simulink library "mec_pointmass_generic_ATvoith_DIWA_NXT"  (R2016a)
settings: Solver=ode45  SolverMode=SingleTasking  StartTime=0.0  StopTime=10.0  RelTol=1e-3
undefined symbols (not defined in the file): sMP
(part 2 of 4)

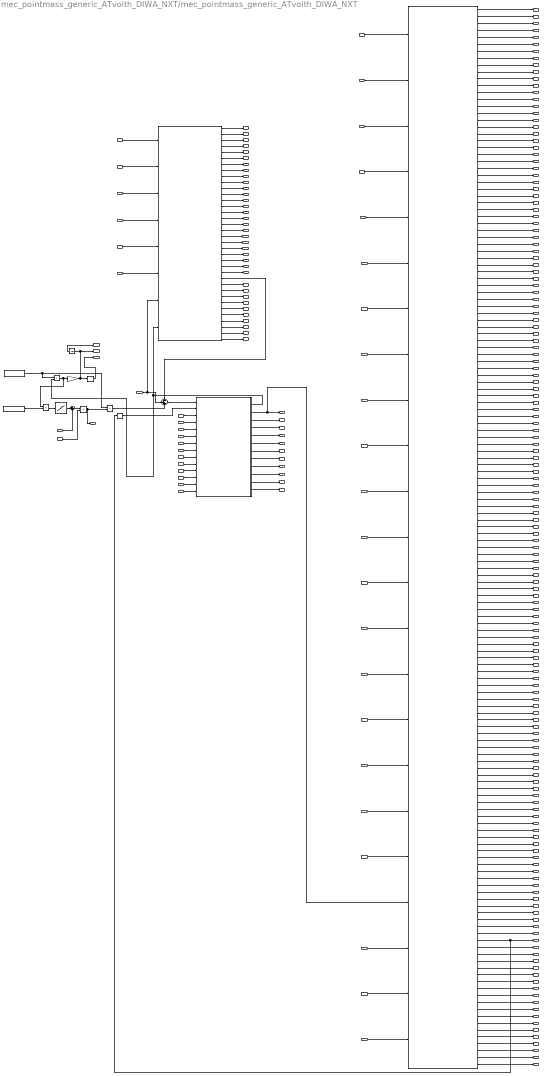
== system mec_pointmass_generic_ATvoith_DIWA_NXT/mec_pointmass_generic_ATvoith_DIWA_NXT  ==
  tcm_AKc2 : Inport
  mec_eng_CrankMean_torque : Inport  Port=2
  tcm_p_EK : Inport  Port=3
  tcm_p_DK : Inport  Port=4
  tcm_p_SK : Inport  Port=5
  tcm_p_PB : Inport  Port=6
  tcm_p_TWB : Inport  Port=7
  tcm_p_TGB : Inport  Port=8
  tcm_AKs2 : Inport  Port=9
  cpc_cdA_offset : Inport  Port=10
  env_curv_pm : Inport  Port=11
  env_density : Inport  Port=12
  env_road_slope_pct : Inport  Port=13
  mec_brk_Axle1_left_torque : Inport  Port=14
  mec_brk_Axle1_right_torque : Inport  Port=15
  mec_brk_Axle2_left_torque : Inport  Port=16
  mec_brk_Axle2_right_torque : Inport  Port=17
  mec_brk_Axle3_left_torque : Inport  Port=18
  mec_brk_Axle3_right_torque : Inport  Port=19
  mec_brk_Axle4_left_torque : Inport  Port=20
  mec_brk_Axle4_right_torque : Inport  Port=21
  mec_brk_TrailerAxle1_left_torque : Inport  Port=22
  mec_brk_TrailerAxle1_right_torque : Inport  Port=23
  mec_brk_TrailerAxle2_left_torque : Inport  Port=24
  mec_brk_TrailerAxle2_right_torque : Inport  Port=25
  mec_brk_TrailerAxle3_left_torque : Inport  Port=26
  mec_brk_TrailerAxle3_right_torque : Inport  Port=27
  mec_ret_Retarder_torque : Inport  Port=28
  mec_veh_GenericLoss_force : Inport  Port=29
  mec_wheel_GenericLoss_torque : Inport  Port=30
  mcm_starter_on : Inport  Port=31
  mec_eng_Starter_torque : Inport  Port=32
  mec_brk_AirCompressor_torque : Inport  Port=33
  mec_eng_Generator_torque : Inport  Port=34
  mec_eng_Consumer_torque : Inport  Port=35
  mec_eng_MainFan_torque : Inport  Port=36
  mec_eng_MainPump_torque : Inport  Port=37
  mec_eng_EmotCrankshaft_torque : Inport  Port=38
  tcm_p_RGK : Inport  Port=39
  pt_RetTrq_Rq_PT : Inport  Port=40
  tcm_gearAct : Inport  Port=41
  pt_ReqGr_Stat_PT : Inport  Port=42
  env_load_massdiff : Inport  Port=43
  Constant : Constant  Value=scalAngVelStarter
  Constant1 : Constant  Value=iStarter
  DIWA_NXT : Subsystem  mask{DIWA_BB_ParNames=sMP.phys.mec.tx.DIWA_BB_ParNames, DIWA_BB_ParValues=sMP.phys.mec.tx.DIWA_BB_ParValues}
  Derivative2 : Derivative
  Engine : Subsystem
  Gain1 : Gain  Gain=pi/30
  Integrator : Integrator
  Memory : Memory
  Product{,1..3} (4 alike) : Product
  StarterMap : Lookup_n-D  NumberOfTableDimensions=1  BreakpointsForDimension1=[0,2.7027,64.8648,150.4214,260.724,378.378,520.398,657.98,819.858,982.04,1178.378,1286.486,1430.18,1578.378,1789.894,2054.06,2177.6,2616.22,3124.32,3697.3,3757.62]  Table=[319.835,318.919,297.838,271.351,244.364,217.585,191.073,165.144,136.757,109.189,82.9584,69.8576,56.7568,44.1906,32.1593,19.8695,15.6757,7.2814,3.27928,0,0]  InternalRulePriority=Speed  RndMeth=Simplest  InputSameDT=on
  Sum : Sum  Inputs=|++
  Sum1 : Sum  Inputs=-++
  mec_pointmass_generic_ATvoith_std : Subsystem  mask{s1=sMP.phys.mec.settings_iMode, s2=sMP.phys.mec.settings_dt, initCmd='Parameters_mec_pointmass_generic_ATvoith_std_sf', p1=sMP.phys.mec.axle1.iDiff, p2=sMP.phys.mec.axle1.isDriven, p3=sMP.phys.mec.axle1.isRearAxle, p4=sMP.phys.mec.brk1.JBrakeDisc_kgm2, p5=sMP.phys.mec.brk1.JHub_kgm2, p6=sMP.phys.mec.axle1.JSideShft_kgm2, p7=sMP.phys.mec.axle2.iDiff, p8=sMP.phys.mec.axle2.isDriven, p9=sMP.phys.mec.axle2.isRearAxle, p10=sMP.phys.mec.brk2.JBrakeDisc_kgm2, p11=sMP.phys.mec.brk2.JHub_kgm2, p12=sMP.phys.mec.axle2.JSideShft_kgm2, p13=sMP.phys.mec.axle3.iDiff, p14=sMP.phys.mec.axle3.isDriven, p15=sMP.phys.mec.axle3.isRearAxle, p16=sMP.phys.mec.brk3.JBrakeDisc_kgm2, p17=sMP.phys.mec.brk3.JHub_kgm2, p18=sMP.phys.mec.axle3.JSideShft_kgm2, p19=sMP.phys.mec.axle4.iDiff, p20=sMP.phys.mec.axle4.isDriven, p21=sMP.phys.mec.axle4.isRearAxle, p22=sMP.phys.mec.brk4.JBrakeDisc_kgm2, p23=sMP.phys.mec.brk4.JHub_kgm2, p24=sMP.phys.mec.axle4.JSideShft_kgm2, p25=sMP.phys.mec.in.cpc_cdA_offset, p26=sMP.phys.mec.in.env_curv_pm, p27=sMP.phys.mec.in.env_density, p28=sMP.phys.mec.in.env_load_massdiff, p29=sMP.phys.mec.in.env_road_slope_pct, p30=sMP.phys.mec.out.mec_brk_Axle1_angAcc, p31=sMP.phys.mec.out.mec_brk_Axle1_angPos, p32=sMP.phys.mec.out.mec_brk_Axle1_angVel, p33=sMP.phys.mec.out.mec_brk_Axle1_left_angAcc, p34=sMP.phys.mec.out.mec_brk_Axle1_left_angPos, p35=sMP.phys.mec.out.mec_brk_Axle1_left_angVel, p36=sMP.phys.mec.in.mec_brk_Axle1_left_torque, p37=sMP.phys.mec.out.mec_brk_Axle1_right_angAcc, p38=sMP.phys.mec.out.mec_brk_Axle1_right_angPos, p39=sMP.phys.mec.out.mec_brk_Axle1_right_angVel, p40=sMP.phys.mec.in.mec_brk_Axle1_right_torque, p41=sMP.phys.mec.out.mec_brk_Axle2_angAcc, p42=sMP.phys.mec.out.mec_brk_Axle2_angPos, p43=sMP.phys.mec.out.mec_brk_Axle2_angVel, p44=sMP.phys.mec.out.mec_brk_Axle2_left_angAcc, p45=sMP.phys.mec.out.mec_brk_Axle2_left_angPos, p46=sMP.phys.mec.out.mec_brk_Axle2_left_angVel, p47=sMP.phys.mec.in.mec_brk_Axle2_left_torque, p48=sMP.phys.mec.out.mec_brk_Axle2_right_angAcc, p49=sMP.phys.mec.out.mec_brk_Axle2_right_angPos, p50=sMP.phys.mec.out.mec_brk_Axle2_right_angVel, p51=sMP.phys.mec.in.mec_brk_Axle2_right_torque, p52=sMP.phys.mec.out.mec_brk_Axle3_angAcc, p53=sMP.phys.mec.out.mec_brk_Axle3_angPos, p54=sMP.phys.mec.out.mec_brk_Axle3_angVel, p55=sMP.phys.mec.out.mec_brk_Axle3_left_angAcc, p56=sMP.phys.mec.out.mec_brk_Axle3_left_angPos, p57=sMP.phys.mec.out.mec_brk_Axle3_left_angVel, p58=sMP.phys.mec.in.mec_brk_Axle3_left_torque, p59=sMP.phys.mec.out.mec_brk_Axle3_right_angAcc, p60=sMP.phys.mec.out.mec_brk_Axle3_right_angPos, p61=sMP.phys.mec.out.mec_brk_Axle3_right_angVel, p62=sMP.phys.mec.in.mec_brk_Axle3_right_torque, p63=sMP.phys.mec.out.mec_brk_Axle4_angAcc, p64=sMP.phys.mec.out.mec_brk_Axle4_angPos, p65=sMP.phys.mec.out.mec_brk_Axle4_angVel, p66=sMP.phys.mec.out.mec_brk_Axle4_left_angAcc, p67=sMP.phys.mec.out.mec_brk_Axle4_left_angPos, p68=sMP.phys.mec.out.mec_brk_Axle4_left_angVel, p69=sMP.phys.mec.in.mec_brk_Axle4_left_torque, p70=sMP.phys.mec.out.mec_brk_Axle4_right_angAcc, p71=sMP.phys.mec.out.mec_brk_Axle4_right_angPos, p72=sMP.phys.mec.out.mec_brk_Axle4_right_angVel, p73=sMP.phys.mec.in.mec_brk_Axle4_right_torque, p74=sMP.phys.mec.out.mec_brk_TrailerAxle1_angAcc, p75=sMP.phys.mec.out.mec_brk_TrailerAxle1_angPos, p76=sMP.phys.mec.out.mec_brk_TrailerAxle1_angVel, p77=sMP.phys.mec.out.mec_brk_TrailerAxle1_left_angAcc, p78=sMP.phys.mec.out.mec_brk_TrailerAxle1_left_angPos, p79=sMP.phys.mec.out.mec_brk_TrailerAxle1_left_angVel, p80=sMP.phys.mec.in.mec_brk_TrailerAxle1_left_torque, p81=sMP.phys.mec.out.mec_brk_TrailerAxle1_right_angAcc, p82=sMP.phys.mec.out.mec_brk_TrailerAxle1_right_angPos, p83=sMP.phys.mec.out.mec_brk_TrailerAxle1_right_angVel, p84=sMP.phys.mec.in.mec_brk_TrailerAxle1_right_torque, p85=sMP.phys.mec.out.mec_brk_TrailerAxle2_angAcc, p86=sMP.phys.mec.out.mec_brk_TrailerAxle2_angPos, p87=sMP.phys.mec.out.mec_brk_TrailerAxle2_angVel, p88=sMP.phys.mec.out.mec_brk_TrailerAxle2_left_angAcc, p89=sMP.phys.mec.out.mec_brk_TrailerAxle2_left_angPos, p90=sMP.phys.mec.out.mec_brk_TrailerAxle2_left_angVel, p91=sMP.phys.mec.in.mec_brk_TrailerAxle2_left_torque, p92=sMP.phys.mec.out.mec_brk_TrailerAxle2_right_angAcc, p93=sMP.phys.mec.out.mec_brk_TrailerAxle2_right_angPos, p94=sMP.phys.mec.out.mec_brk_TrailerAxle2_right_angVel, p95=sMP.phys.mec.in.mec_brk_TrailerAxle2_right_torque, p96=sMP.phys.mec.out.mec_brk_TrailerAxle3_angAcc, p97=sMP.phys.mec.out.mec_brk_TrailerAxle3_angPos, p98=sMP.phys.mec.out.mec_brk_TrailerAxle3_angVel, p99=sMP.phys.mec.out.mec_brk_TrailerAxle3_left_angAcc, p100=sMP.phys.mec.out.mec_brk_TrailerAxle3_left_angPos, p101=sMP.phys.mec.out.mec_brk_TrailerAxle3_left_angVel, p102=sMP.phys.mec.in.mec_brk_TrailerAxle3_left_torque, p103=sMP.phys.mec.out.mec_brk_TrailerAxle3_right_angAcc, p104=sMP.phys.mec.out.mec_brk_TrailerAxle3_right_angPos, p105=sMP.phys.mec.out.mec_brk_TrailerAxle3_right_angVel, p106=sMP.phys.mec.in.mec_brk_TrailerAxle3_right_torque, p107=sMP.phys.mec.in.mec_eng_CrankMean_torque, p108=sMP.phys.mec.out.mec_ret_Retarder_angAcc, p109=sMP.phys.mec.out.mec_ret_Retarder_angPos, p110=sMP.phys.mec.out.mec_ret_Retarder_angVel, p111=sMP.phys.mec.in.mec_ret_Retarder_torque, p112=sMP.phys.mec.out.mec_tx_inclRoadSns, p113=sMP.phys.mec.out.mec_tx_nGbOutD3Sns, p114=sMP.phys.mec.out.mec_tx_nGbOutDzAwSns, p115=sMP.phys.mec.out.mec_tx_nGbOutDzSfSns, p116=sMP.phys.mec.out.mec_tx_nGbOutDzTuAwSns, p117=sMP.phys.mec.out.mec_tx_nGbOutSns, p118=sMP.phys.mec.out.mec_veh_AxleLoad1, p119=sMP.phys.mec.out.mec_veh_AxleLoad2, p120=sMP.phys.mec.out.mec_veh_AxleLoad3, p121=sMP.phys.mec.out.mec_veh_AxleLoad4, p122=sMP.phys.mec.out.mec_veh_fRollCoeffOverall, p123=sMP.phys.mec.in.mec_veh_GenericLoss_force, p124=sMP.phys.mec.out.mec_veh_GenericLoss_transAcc, p125=sMP.phys.mec.out.mec_veh_GenericLoss_transPos, p126=sMP.phys.mec.out.mec_veh_GenericLoss_transVel, p127=sMP.phys.mec.out.mec_veh_massVehicle, p128=sMP.phys.mec.out.mec_veh_Payload, p129=sMP.phys.mec.out.mec_veh_TotalGroCombWeight, p130=sMP.phys.mec.out.mec_veh_TrailerAxleLoad1, p131=sMP.phys.mec.out.mec_veh_TrailerAxleLoad2, p132=sMP.phys.mec.out.mec_veh_TrailerAxleLoad3, p133=sMP.phys.mec.out.mec_veh_transAcc, p134=sMP.phys.mec.out.mec_veh_transPos, p135=sMP.phys.mec.out.mec_veh_transVel, p136=sMP.phys.mec.out.mec_veh_VehVelReferenceCool_velocity, p137=sMP.phys.mec.out.mec_veh_VehVelReferenceUhood_velocity, p138=sMP.phys.mec.out.mec_wheel_GenericLoss_angAcc, p139=sMP.phys.mec.out.mec_wheel_GenericLoss_angPos, p140=sMP.phys.mec.out.mec_wheel_GenericLoss_angVel, p141=sMP.phys.mec.in.mec_wheel_GenericLoss_torque, p142=sMP.phys.mec.out.mec_brk_Axle1_omBrk_info, p143=sMP.phys.mec.out.mec_brk_Axle1_omIn_info, p144=sMP.phys.mec.out.mec_brk_Axle1_TiBrk_info, p145=sMP.phys.mec.out.mec_brk_Axle1_TiLoss_info, p146=sMP.phys.mec.out.mec_brk_Axle1_TIn_info, p147=sMP.phys.mec.out.mec_brk_Axle2_omIn_info, p148=sMP.phys.mec.out.mec_brk_Axle2_TiBrk_info, p149=sMP.phys.mec.out.mec_brk_Axle2_TiLoss_info, p150=sMP.phys.mec.out.mec_brk_Axle2_TIn_info, p151=sMP.phys.mec.out.mec_brk_Axle3_omIn_info, p152=sMP.phys.mec.out.mec_brk_Axle3_TiBrk_info, p153=sMP.phys.mec.out.mec_brk_Axle3_TiLoss_info, p154=sMP.phys.mec.out.mec_brk_Axle3_TIn_info, p155=sMP.phys.mec.out.mec_brk_Axle4_omIn_info, p156=sMP.phys.mec.out.mec_brk_Axle4_TiBrk_info, p157=sMP.phys.mec.out.mec_brk_Axle4_TiLoss_info, p158=sMP.phys.mec.out.mec_brk_Axle4_TIn_info, p159=sMP.phys.mec.out.mec_brk_TrailerAxle1_omIn_info, p160=sMP.phys.mec.out.mec_brk_TrailerAxle1_TiBrk_info, p161=sMP.phys.mec.out.mec_brk_TrailerAxle1_TiLoss_info, p162=sMP.phys.mec.out.mec_brk_TrailerAxle1_TIn_info, p163=sMP.phys.mec.out.mec_brk_TrailerAxle2_omIn_info, p164=sMP.phys.mec.out.mec_brk_TrailerAxle2_TiBrk_info, p165=sMP.phys.mec.out.mec_brk_TrailerAxle2_TiLoss_info, p166=sMP.phys.mec.out.mec_brk_TrailerAxle2_TIn_info, p167=sMP.phys.mec.out.mec_brk_TrailerAxle3_omIn_info, p168=sMP.phys.mec.out.mec_brk_TrailerAxle3_TiBrk_info, p169=sMP.phys.mec.out.mec_brk_TrailerAxle3_TiLoss_info, p170=sMP.phys.mec.out.mec_brk_TrailerAxle3_TIn_info, p171=sMP.phys.mec.out.mec_brk_TrailerWheel1_TiLossRollRes_info, p172=sMP.phys.mec.out.mec_brk_TrailerWheel2_TiLossRollRes_info, p173=sMP.phys.mec.out.mec_brk_TrailerWheel3_TiLossRollRes_info, p174=sMP.phys.mec.out.mec_brk_Wheel1_TiLossRollRes_info, p175=sMP.phys.mec.out.mec_brk_Wheel2_TiLossRollRes_info, p176=sMP.phys.mec.out.mec_brk_Wheel3_TiLossRollRes_info, p177=sMP.phys.mec.out.mec_brk_Wheel4_TiLossRollRes_info, p178=sMP.phys.mec.out.mec_ret_T_info, p179=sMP.phys.mec.out.mec_sht_omShtF_info, p180=sMP.phys.mec.out.mec_sht_omShtR_info, p181=sMP.phys.mec.out.mec_sht_TiLossShtF_info, p182=sMP.phys.mec.out.mec_sht_TiLossShtR_info, p183=sMP.phys.mec.out.mec_tfc_omOut_info, p184=sMP.phys.mec.out.mec_tfc_TiLoss_info, p185=sMP.phys.mec.out.mec_tfc_TOutFront_info, p186=sMP.phys.mec.out.mec_tfc_TOutRear_info, p187=sMP.phys.mec.out.mec_veh_domFW_info, p188=sMP.phys.mec.out.mec_veh_dphiFW_info, p189=sMP.phys.mec.out.mec_veh_FiAirDrag_info, p190=sMP.phys.mec.out.mec_veh_FiGradeRes_info, p191=sMP.phys.mec.out.mec_veh_FWheelTraction_info, p192=sMP.phys.mec.out.mec_veh_sFW_info, p193=sMP.phys.mec.out.mec_veh_TiFW_info, p194=sMP.phys.mec.out.mec_veh_vehConfig_info, p195=sMP.phys.mec.out.mec_wheel_Axle1_T_info, p196=sMP.phys.mec.out.mec_wheel_Axle2_T_info, p197=sMP.phys.mec.out.mec_wheel_Axle3_T_info, p198=sMP.phys.mec.out.mec_wheel_Axle4_T_info, p199=sMP.phys.mec.out.mec_wheel_TrailerAxle1_T_info, p200=sMP.phys.mec.out.mec_wheel_TrailerAxle2_T_info, p201=sMP.phys.mec.out.mec_wheel_TrailerAxle3_T_info, p202=sMP.phys.mec.shtF.JPropShaft_kgm2, p203=sMP.phys.mec.shtR.JPropShaft_kgm2, p204=sMP.phys.mec.ret.iRet, p205=sMP.phys.mec.ret.JRet_kgm2, p206=sMP.phys.mec.ret.JRetdrvgear_kgm2, p207=sMP.phys.mec.trailerAxle1.iDiff, p208=sMP.phys.mec.trailerAxle1.isDriven, p209=sMP.phys.mec.trailerAxle1.isRearAxle, p210=sMP.phys.mec.trailerBrk1.JBrakeDisc_kgm2, p211=sMP.phys.mec.trailerBrk1.JHub_kgm2, p212=sMP.phys.mec.trailerAxle1.JSideShft_kgm2, p213=sMP.phys.mec.trailerAxle2.iDiff, p214=sMP.phys.mec.trailerAxle2.isDriven, p215=sMP.phys.mec.trailerAxle2.isRearAxle, p216=sMP.phys.mec.trailerBrk2.JBrakeDisc_kgm2, p217=sMP.phys.mec.trailerBrk2.JHub_kgm2, p218=sMP.phys.mec.trailerAxle2.JSideShft_kgm2, p219=sMP.phys.mec.trailerAxle3.iDiff, p220=sMP.phys.mec.trailerAxle3.isDriven, p221=sMP.phys.mec.trailerAxle3.isRearAxle, p222=sMP.phys.mec.trailerBrk3.JBrakeDisc_kgm2, p223=sMP.phys.mec.trailerBrk3.JHub_kgm2, p224=sMP.phys.mec.trailerAxle3.JSideShft_kgm2, p225=sMP.phys.mec.tfc.JTfc_kgm2, p226=sMP.phys.mec.tfc.stTrfGrBoxHi, p227=sMP.phys.mec.aero.aeroCdA_m2, p228=sMP.phys.mec.aero.aeroRhoAirDensity_kgpm3, p229=sMP.phys.mec.massLoad.number_of_weights, p230=sMP.phys.mec.mass.startGCW_kg, p231=sMP.phys.mec.wheel1.fRollCoeff, p232=sMP.phys.mec.wheel1.JWheel_kgm2, p233=sMP.phys.mec.wheel1.rDyn_m, p234=sMP.phys.mec.wheel2.fRollCoeff, p235=sMP.phys.mec.wheel2.JWheel_kgm2, p236=sMP.phys.mec.wheel2.rDyn_m, p237=sMP.phys.mec.wheel3.fRollCoeff, p238=sMP.phys.mec.wheel3.JWheel_kgm2, p239=sMP.phys.mec.wheel3.rDyn_m, p240=sMP.phys.mec.wheel4.fRollCoeff, p241=sMP.phys.mec.wheel4.JWheel_kgm2, p242=sMP.phys.mec.wheel4.rDyn_m, p243=sMP.phys.mec.trailerWheel1.fRollCoeff, p244=sMP.phys.mec.trailerWheel1.JWheel_kgm2, p245=sMP.phys.mec.trailerWheel1.rDyn_m, p246=sMP.phys.mec.trailerWheel2.fRollCoeff, p247=sMP.phys.mec.trailerWheel2.JWheel_kgm2, p248=sMP.phys.mec.trailerWheel2.rDyn_m, p249=sMP.phys.mec.trailerWheel3.fRollCoeff, p250=sMP.phys.mec.trailerWheel3.JWheel_kgm2, p251=sMP.phys.mec.trailerWheel3.rDyn_m, p252=sMP.phys.mec.mecConsumers.genericWheelLoss_dim, p253=sMP.phys.mec.mecConsumers.genericVehicleLoss_dim, p254=sMP.phys.mec.axle1.axleLoss_dim, p255=sMP.phys.mec.axle1.axleLoss_map_torqueAxleIn_Nm, p256=sMP.phys.mec.axle1.axleLoss_x_speedAxleOut_rpm, p257=sMP.phys.mec.axle1.axleLoss_y_torqueAxleIn_Nm, p258=sMP.phys.mec.axle2.axleLoss_dim, p259=sMP.phys.mec.axle2.axleLoss_map_torqueAxleIn_Nm, p260=sMP.phys.mec.axle2.axleLoss_x_speedAxleOut_rpm, p261=sMP.phys.mec.axle2.axleLoss_y_torqueAxleIn_Nm, p262=sMP.phys.mec.axle3.axleLoss_dim, p263=sMP.phys.mec.axle3.axleLoss_map_torqueAxleIn_Nm, p264=sMP.phys.mec.axle3.axleLoss_x_speedAxleOut_rpm, p265=sMP.phys.mec.axle3.axleLoss_y_torqueAxleIn_Nm, p266=sMP.phys.mec.axle4.axleLoss_dim, p267=sMP.phys.mec.axle4.axleLoss_map_torqueAxleIn_Nm, p268=sMP.phys.mec.axle4.axleLoss_x_speedAxleOut_rpm, p269=sMP.phys.mec.axle4.axleLoss_y_torqueAxleIn_Nm, p270=sMP.phys.mec.shtF.shtLoss_dim, p271=sMP.phys.mec.shtF.shtLoss_map_torqueShtIn_Nm, p272=sMP.phys.mec.shtF.shtLoss_x_speedShtIn_rpm, p273=sMP.phys.mec.shtF.shtLoss_y_torqueShtIn_Nm, p274=sMP.phys.mec.shtR.shtLoss_dim, p275=sMP.phys.mec.shtR.shtLoss_map_torqueShtIn_Nm, p276=sMP.phys.mec.shtR.shtLoss_x_speedShtIn_rpm, p277=sMP.phys.mec.shtR.shtLoss_y_torqueShtIn_Nm, p278=sMP.phys.mec.trailerAxle1.axleLoss_dim, p279=sMP.phys.mec.trailerAxle1.axleLoss_map_torqueAxleIn_Nm, p280=sMP.phys.mec.trailerAxle1.axleLoss_x_speedAxleOut_rpm, p281=sMP.phys.mec.trailerAxle1.axleLoss_y_torqueAxleIn_Nm, p282=sMP.phys.mec.trailerAxle2.axleLoss_dim, p283=sMP.phys.mec.trailerAxle2.axleLoss_map_torqueAxleIn_Nm, p284=sMP.phys.mec.trailerAxle2.axleLoss_x_speedAxleOut_rpm, p285=sMP.phys.mec.trailerAxle2.axleLoss_y_torqueAxleIn_Nm, p286=sMP.phys.mec.trailerAxle3.axleLoss_dim, p287=sMP.phys.mec.trailerAxle3.axleLoss_map_torqueAxleIn_Nm, p288=sMP.phys.mec.trailerAxle3.axleLoss_x_speedAxleOut_rpm, p289=sMP.phys.mec.trailerAxle3.axleLoss_y_torqueAxleIn_Nm, p290=sMP.phys.mec.tfc.iTfc, p291=sMP.phys.mec.tfc.tfcLoss_dim, p292=sMP.phys.mec.tfc.tfcLoss_map_torqueTfcIn_Nm, p293=sMP.phys.mec.tfc.tfcLoss_x_speedTfcIn_rpm, p294=sMP.phys.mec.tfc.tfcLoss_y_torqueTfcIn_Nm, p295=sMP.phys.mec.tfc.torqueDistribution, p296=sMP.phys.mec.massLoad.mass_distribution, p297=sMP.phys.mec.mecConsumers.genericWheelLoss_x_speed_rpm, p298=sMP.phys.mec.mecConsumers.genericWheelLoss_map_lossTorque_Nm, p299=sMP.phys.mec.mecConsumers.genericVehicleLoss_x_velocity_kmh, p300=sMP.phys.mec.mecConsumers.genericVehicleLoss_map_loss_N}
      mask prompts: s1 "Solver Type: settings_iMode [-]"; s2 "Solver Step Size: settings_dt [s]"; initCmd "Initialization command"; p1 "Ratio Differential Gear [-] export=true name=iDiff prio=1 dataSetName=axle_dummy dataClassType=axle dataClassName=$dataClassNameAxle$ moduleXmlReference=$moduleXmlReferenceAxle$ unit='-' description='Ratio Differential Gear': axle1.iDiff [-]"; p2 "Is driven Axle? [-] export=true name=isDriven prio=1 dataSetName=axle_dummy dataClassType=axle dataClassName=$dataClassNameAxle$ moduleXmlReference=$moduleXmlReferenceAxle$ unit='-' description='Is Driven Axle': axle1.isDriven [-]"; p3 "Is rear Axle? [-] export=true name=isRearAxle prio=1 dataSetName=axle_dummy dataClassType=axle dataClassName=$dataClassNameAxle$ moduleXmlReference=$moduleXmlReferenceAxle$ unit='-' description='Is Rear Axle': axle1.isRearAxle [-]"; p4 "Inertia Brake Disc  [kgm^2] export=true name=JBrakeDisc_kgm2 prio=1 dataSetName=brk_dummy dataClassType=brk dataClassName=$dataClassNameBrk$ moduleXmlReference=$moduleXmlReferenceBrk$ unit='kgm^2' description='Inertia Brake Disc': axle1.JBrakeDisc_kgm2 [kgm²]"; p5 "Inertia Hub  [kgm^2] export=true name=JHub_kgm2 prio=1 dataSetName=brk_dummy dataClassType=brk dataClassName=$dataClassNameBrk$ moduleXmlReference=$moduleXmlReferenceBrk$ unit='kgm^2' description='Inertia Hub': axle1.JHub_kgm2 [-]"; p6 "Inertia Side Shaft [kgm^2] export=true name=JSideShft_kgm2 prio=1 dataSetName=axle_dummy dataClassType=axle dataClassName=$dataClassNameAxle$ moduleXmlReference=$moduleXmlReferenceAxle$ unit='kgm^2' description='Inertia Side Shaft': axle1.JSideShft_kgm2 [kgm²]"; p7 "Ratio Differential Gear [-] export=true name=iDiff prio=1 dataSetName=axle_dummy dataClassType=axle dataClassName=$dataClassNameAxle$ moduleXmlReference=$moduleXmlReferenceAxle$ unit='-' description='Ratio Differential Gear': axle2.iDiff [-]"; p8 "Is driven Axle? [-] export=true name=isDriven prio=1 dataSetName=axle_dummy dataClassType=axle dataClassName=$dataClassNameAxle$ moduleXmlReference=$moduleXmlReferenceAxle$ unit='-' description='Is Driven Axle': axle2.isDriven [-]"; p9 "Is rear Axle? [-] export=true name=isRearAxle prio=1 dataSetName=axle_dummy dataClassType=axle dataClassName=$dataClassNameAxle$ moduleXmlReference=$moduleXmlReferenceAxle$ unit='-' description='Is Rear Axle': axle2.isRearAxle [-]"; p10 "Inertia Brake Disc  [kgm^2] export=true name=JBrakeDisc_kgm2 prio=1 dataSetName=brk_dummy dataClassType=brk dataClassName=$dataClassNameBrk$ moduleXmlReference=$moduleXmlReferenceBrk$ unit='kgm^2' description='Inertia Brake Disc': axle2.JBrakeDisc_kgm2 [kgm²]"; p11 "Inertia Hub  [kgm^2] export=true name=JHub_kgm2 prio=1 dataSetName=brk_dummy dataClassType=brk dataClassName=$dataClassNameBrk$ moduleXmlReference=$moduleXmlReferenceBrk$ unit='kgm^2' description='Inertia Hub': axle2.JHub_kgm2 [-]"; p12 "Inertia Side Shaft [kgm^2] export=true name=JSideShft_kgm2 prio=1 dataSetName=axle_dummy dataClassType=axle dataClassName=$dataClassNameAxle$ moduleXmlReference=$moduleXmlReferenceAxle$ unit='kgm^2' description='Inertia Side Shaft': axle2.JSideShft_kgm2 [kgm²]"; p13 "Ratio Differential Gear [-] export=true name=iDiff prio=1 dataSetName=axle_dummy dataClassType=axle dataClassName=$dataClassNameAxle$ moduleXmlReference=$moduleXmlReferenceAxle$ unit='-' description='Ratio Differential Gear': axle3.iDiff [-]"; p14 "Is driven Axle? [-] export=true name=isDriven prio=1 dataSetName=axle_dummy dataClassType=axle dataClassName=$dataClassNameAxle$ moduleXmlReference=$moduleXmlReferenceAxle$ unit='-' description='Is Driven Axle': axle3.isDriven [-]"; p15 "Is rear Axle? [-] export=true name=isRearAxle prio=1 dataSetName=axle_dummy dataClassType=axle dataClassName=$dataClassNameAxle$ moduleXmlReference=$moduleXmlReferenceAxle$ unit='-' description='Is Rear Axle': axle3.isRearAxle [-]"; p16 "Inertia Brake Disc  [kgm^2] export=true name=JBrakeDisc_kgm2 prio=1 dataSetName=brk_dummy dataClassType=brk dataClassName=$dataClassNameBrk$ moduleXmlReference=$moduleXmlReferenceBrk$ unit='kgm^2' description='Inertia Brake Disc': axle3.JBrakeDisc_kgm2 [kgm²]"; p17 "Inertia Hub  [kgm^2] export=true name=JHub_kgm2 prio=1 dataSetName=brk_dummy dataClassType=brk dataClassName=$dataClassNameBrk$ moduleXmlReference=$moduleXmlReferenceBrk$ unit='kgm^2' description='Inertia Hub': axle3.JHub_kgm2 [-]"; p18 "Inertia Side Shaft [kgm^2] export=true name=JSideShft_kgm2 prio=1 dataSetName=axle_dummy dataClassType=axle dataClassName=$dataClassNameAxle$ moduleXmlReference=$moduleXmlReferenceAxle$ unit='kgm^2' description='Inertia Side Shaft': axle3.JSideShft_kgm2 [kgm²]"; p19 "Ratio Differential Gear [-] export=true name=iDiff prio=1 dataSetName=axle_dummy dataClassType=axle dataClassName=$dataClassNameAxle$ moduleXmlReference=$moduleXmlReferenceAxle$ unit='-' description='Ratio Differential Gear': axle4.iDiff [-]"; p20 "Is driven Axle? [-] export=true name=isDriven prio=1 dataSetName=axle_dummy dataClassType=axle dataClassName=$dataClassNameAxle$ moduleXmlReference=$moduleXmlReferenceAxle$ unit='-' description='Is Driven Axle': axle4.isDriven [-]"; p21 "Is rear Axle? [-] export=true name=isRearAxle prio=1 dataSetName=axle_dummy dataClassType=axle dataClassName=$dataClassNameAxle$ moduleXmlReference=$moduleXmlReferenceAxle$ unit='-' description='Is Rear Axle': axle4.isRearAxle [-]"; p22 "Inertia Brake Disc  [kgm^2] export=true name=JBrakeDisc_kgm2 prio=1 dataSetName=brk_dummy dataClassType=brk dataClassName=$dataClassNameBrk$ moduleXmlReference=$moduleXmlReferenceBrk$ unit='kgm^2' description='Inertia Brake Disc': axle4.JBrakeDisc_kgm2 [kgm²]"; p23 "Inertia Hub  [kgm^2] export=true name=JHub_kgm2 prio=1 dataSetName=brk_dummy dataClassType=brk dataClassName=$dataClassNameBrk$ moduleXmlReference=$moduleXmlReferenceBrk$ unit='kgm^2' description='Inertia Hub': axle4.JHub_kgm2 [-]"; p24 "Inertia Side Shaft [kgm^2] export=true name=JSideShft_kgm2 prio=1 dataSetName=axle_dummy dataClassType=axle dataClassName=$dataClassNameAxle$ moduleXmlReference=$moduleXmlReferenceAxle$ unit='kgm^2' description='Inertia Side Shaft': axle4.JSideShft_kgm2 [kgm²]"; p25 "Additive Controlable Air Resistance (init) export=$sw_cpc_cdA_offset$ name=cpc_cdA_offset prio=1 dataSetName=std dataClassType=initIO dataClassName=initIO unit='' description='Additive Controlable Air Resistance': interface_IO.cpc_cdA_offset_0 [-]"; p26 "Curve Curvature (init) export=$sw_env_curv_pm$ name=env_curv_pm prio=1 dataSetName=std dataClassType=initIO dataClassName=initIO unit='1/m' description='Curve Curvature': interface_IO.env_curv_pm_0 [-]"; p27 "Air density from environment (init) export=$sw_env_density$ name=env_density prio=1 dataSetName=std dataClassType=initIO dataClassName=initIO unit='kg/m^3' description='Air density from environment': interface_IO.env_density_0 [-]"; p28 "Mass Difference (init) export=$sw_env_load_massdiff$ name=env_load_massdiff prio=1 dataSetName=std dataClassType=initIO dataClassName=initIO unit='1/m' description='Curve Curvature': interface_IO.env_load_massdiff_0 [-]"; p29 "Slope of road from environment (init) export=$sw_env_road_slope_pct$ name=env_road_slope_pct prio=1 dataSetName=std dataClassType=initIO dataClassName=initIO unit='-' description='Slope of road from environment': interface_IO.env_road_slope_pct_0 [-]"; p30 "Acceleration Brake 1 (init) export=$sw_mec_brk_Axle1_angAcc$ name=mec_brk_Axle1_angAcc prio=1 dataSetName=std dataClassType=initIO dataClassName=initIO unit='rad/s^2' description='Acceleration Brake 1': interface_IO.mec_brk_Axle1_angAcc_0 [-]"; p31 "Angle Brake 1 (init) export=$sw_mec_brk_Axle1_angPos$ name=mec_brk_Axle1_angPos prio=1 dataSetName=std dataClassType=initIO dataClassName=initIO unit='rad' description='Angle Brake 1': interface_IO.mec_brk_Axle1_angPos_0 [-]"; p32 "Velocity Brake 1 (init) export=$sw_mec_brk_Axle1_angVel$ name=mec_brk_Axle1_angVel prio=1 dataSetName=std dataClassType=initIO dataClassName=initIO unit='rad/s' description='Velocity Brake 1': interface_IO.mec_brk_Axle1_angVel_0 [-]"; p33 "Acceleration Brake 1 left Wheel (init) export=$sw_mec_brk_Axle1_left_angAcc$ name=mec_brk_Axle1_left_angAcc prio=1 dataSetName=std dataClassType=initIO dataClassName=initIO unit='rad/s^2' description='Acceleration Brake 1 left Wheel': interface_IO.mec_brk_Axle1_left_angAcc_0 [-]"; p34 "Angle Brake 1 left Wheel (init) export=$sw_mec_brk_Axle1_left_angPos$ name=mec_brk_Axle1_left_angPos prio=1 dataSetName=std dataClassType=initIO dataClassName=initIO unit='rad' description='Angle Brake 1 left Wheel': interface_IO.mec_brk_Axle1_left_angPos_0 [-]"; p35 "Velocity Brake 1 left Wheel (init) export=$sw_mec_brk_Axle1_left_angVel$ name=mec_brk_Axle1_left_angVel prio=1 dataSetName=std dataClassType=initIO dataClassName=initIO unit='rad/s' description='Velocity Brake 1 left Wheel': interface_IO.mec_brk_Axle1_left_angVel_0 [-]"; p36 "Torque Brake 1 left Wheel (init) export=$sw_mec_brk_Axle1_left_torque$ name=mec_brk_Axle1_left_torque prio=1 dataSetName=std dataClassType=initIO dataClassName=initIO unit='Nm' description='Torque Brake 1 left Wheel': interface_IO.mec_brk_Axle1_left_torque_0 [-]"; p37 "Acceleration Brake 1 right Wheel (init) export=$sw_mec_brk_Axle1_right_angAcc$ name=mec_brk_Axle1_right_angAcc prio=1 dataSetName=std dataClassType=initIO dataClassName=initIO unit='rad/s^2' description='Acceleration Brake 1 right Wheel': interface_IO.mec_brk_Axle1_right_angAcc_0 [-]"; p38 "Angle Brake 1 right Wheel (init) export=$sw_mec_brk_Axle1_right_angPos$ name=mec_brk_Axle1_right_angPos prio=1 dataSetName=std dataClassType=initIO dataClassName=initIO unit='rad' description='Angle Brake 1 right Wheel': interface_IO.mec_brk_Axle1_right_angPos_0 [-]"; p39 "Velocity Brake 1 right Wheel (init) export=$sw_mec_brk_Axle1_right_angVel$ name=mec_brk_Axle1_right_angVel prio=1 dataSetName=std dataClassType=initIO dataClassName=initIO unit='rad/s' description='Velocity Brake 1 right Wheel': interface_IO.mec_brk_Axle1_right_angVel_0 [-]"; p40 "Torque Brake 1 left Wheel (init) export=$sw_mec_brk_Axle1_right_torque$ name=mec_brk_Axle1_right_torque prio=1 dataSetName=std dataClassType=initIO dataClassName=initIO unit='Nm' description='Torque Brake 1 left Wheel': interface_IO.mec_brk_Axle1_right_torque_0 [-]"; p41 "Acceleration Brake 2 (init) export=$sw_mec_brk_Axle2_angAcc$ name=mec_brk_Axle2_angAcc prio=1 dataSetName=std dataClassType=initIO dataClassName=initIO unit='rad/s^2' description='Acceleration Brake 2': interface_IO.mec_brk_Axle2_angAcc_0 [-]"; p42 "Angle Brake 2 (init) export=$sw_mec_brk_Axle2_angPos$ name=mec_brk_Axle2_angPos prio=1 dataSetName=std dataClassType=initIO dataClassName=initIO unit='rad' description='Angle Brake 2': interface_IO.mec_brk_Axle2_angPos_0 [-]"; p43 "Velocity Brake 2 (init) export=$sw_mec_brk_Axle2_angVel$ name=mec_brk_Axle2_angVel prio=1 dataSetName=std dataClassType=initIO dataClassName=initIO unit='rad/s' description='Velocity Brake 3': interface_IO.mec_brk_Axle2_angVel_0 [-]"; p44 "Acceleration Brake 2 left Wheel (init) export=$sw_mec_brk_Axle2_left_angAcc$ name=mec_brk_Axle2_left_angAcc prio=1 dataSetName=std dataClassType=initIO dataClassName=initIO unit='rad/s^2' description='Acceleration Brake 2 left Wheel': interface_IO.mec_brk_Axle2_left_angAcc_0 [-]"; p45 "Angle Brake 2 left Wheel (init) export=$sw_mec_brk_Axle2_left_angPos$ name=mec_brk_Axle2_left_angPos prio=1 dataSetName=std dataClassType=initIO dataClassName=initIO unit='rad' description='Angle Brake 2 left Wheel': interface_IO.mec_brk_Axle2_left_angPos_0 [-]"; p46 "Velocity Brake 2 left Wheel (init) export=$sw_mec_brk_Axle2_left_angVel$ name=mec_brk_Axle2_left_angVel prio=1 dataSetName=std dataClassType=initIO dataClassName=initIO unit='rad/s' description='Velocity Brake 3 left Wheel': interface_IO.mec_brk_Axle2_left_angVel_0 [-]"; p47 "Torque Brake 2 left Wheel (init) export=$sw_mec_brk_Axle2_left_torque$ name=mec_brk_Axle2_left_torque prio=1 dataSetName=std dataClassType=initIO dataClassName=initIO unit='Nm' description='Torque Brake 2 left Wheel': interface_IO.mec_brk_Axle2_left_torque_0 [-]"; p48 "Acceleration Brake 2 right Wheel (init) export=$sw_mec_brk_Axle2_right_angAcc$ name=mec_brk_Axle2_right_angAcc prio=1 dataSetName=std dataClassType=initIO dataClassName=initIO unit='rad/s^2' description='Acceleration Brake 2 right Wheel': interface_IO.mec_brk_Axle2_right_angAcc_0 [-]"; p49 "Angle Brake 2 right Wheel (init) export=$sw_mec_brk_Axle2_right_angPos$ name=mec_brk_Axle2_right_angPos prio=1 dataSetName=std dataClassType=initIO dataClassName=initIO unit='rad' description='Angle Brake 2 right Wheel': interface_IO.mec_brk_Axle2_right_angPos_0 [-]"; p50 "Velocity Brake 2 right Wheel (init) export=$sw_mec_brk_Axle2_right_angVel$ name=mec_brk_Axle2_right_angVel prio=1 dataSetName=std dataClassType=initIO dataClassName=initIO unit='rad/s' description='Velocity Brake 3 right Wheel': interface_IO.mec_brk_Axle2_right_angVel_0 [-]"; p51 "Torque Brake 2 right Wheel (init) export=$sw_mec_brk_Axle2_right_torque$ name=mec_brk_Axle2_right_torque prio=1 dataSetName=std dataClassType=initIO dataClassName=initIO unit='Nm' description='Torque Brake 2 right Wheel': interface_IO.mec_brk_Axle2_right_torque_0 [-]"; p52 "Acceleration Brake 3 (init) export=$sw_mec_brk_Axle3_angAcc$ name=mec_brk_Axle3_angAcc prio=1 dataSetName=std dataClassType=initIO dataClassName=initIO unit='rad/s^2' description='Acceleration Brake 3': interface_IO.mec_brk_Axle3_angAcc_0 [-]"; p53 "Angle Brake 3 (init) export=$sw_mec_brk_Axle3_angPos$ name=mec_brk_Axle3_angPos prio=1 dataSetName=std dataClassType=initIO dataClassName=initIO unit='rad' description='Angle Brake 3': interface_IO.mec_brk_Axle3_angPos_0 [-]"; p54 "Velocity Brake 3 (init) export=$sw_mec_brk_Axle3_angVel$ name=mec_brk_Axle3_angVel prio=1 dataSetName=std dataClassType=initIO dataClassName=initIO unit='rad/s' description='Velocity Brake 3': interface_IO.mec_brk_Axle3_angVel_0 [-]"; p55 "Acceleration Brake 3 left Wheel (init) export=$sw_mec_brk_Axle3_left_angAcc$ name=mec_brk_Axle3_left_angAcc prio=1 dataSetName=std dataClassType=initIO dataClassName=initIO unit='rad/s^2' description='Acceleration Brake 3 left Wheel': interface_IO.mec_brk_Axle3_left_angAcc_0 [-]"; p56 "Angle Brake 3 left Wheel (init) export=$sw_mec_brk_Axle3_left_angPos$ name=mec_brk_Axle3_left_angPos prio=1 dataSetName=std dataClassType=initIO dataClassName=initIO unit='rad' description='Angle Brake 3 left Wheel': interface_IO.mec_brk_Axle3_left_angPos_0 [-]"; p57 "Velocity Brake 3 left Wheel (init) export=$sw_mec_brk_Axle3_left_angVel$ name=mec_brk_Axle3_left_angVel prio=1 dataSetName=std dataClassType=initIO dataClassName=initIO unit='rad/s' description='Velocity Brake 3 left Wheel': interface_IO.mec_brk_Axle3_left_angVel_0 [-]"; p58 "Torque Brake 3 left Wheel (init) export=$sw_mec_brk_Axle3_left_torque$ name=mec_brk_Axle3_left_torque prio=1 dataSetName=std dataClassType=initIO dataClassName=initIO unit='Nm' description='Torque Brake 3 left Wheel': interface_IO.mec_brk_Axle3_left_torque_0 [-]"; p59 "Acceleration Brake 3 right Wheel (init) export=$sw_mec_brk_Axle3_right_angAcc$ name=mec_brk_Axle3_right_angAcc prio=1 dataSetName=std dataClassType=initIO dataClassName=initIO unit='rad/s^2' description='Acceleration Brake 3 right Wheel': interface_IO.mec_brk_Axle3_right_angAcc_0 [-]"; p60 "Angle Brake 3 right Wheel (init) export=$sw_mec_brk_Axle3_right_angPos$ name=mec_brk_Axle3_right_angPos prio=1 dataSetName=std dataClassType=initIO dataClassName=initIO unit='rad' description='Angle Brake 3 right Wheel': interface_IO.mec_brk_Axle3_right_angPos_0 [-]"; p61 "Velocity Brake 3 right Wheel (init) export=$sw_mec_brk_Axle3_right_angVel$ name=mec_brk_Axle3_right_angVel prio=1 dataSetName=std dataClassType=initIO dataClassName=initIO unit='rad/s' description='Velocity Brake 3 right Wheel': interface_IO.mec_brk_Axle3_right_angVel_0 [-]"; p62 "Torque Brake 3 right Wheel (init) export=$sw_mec_brk_Axle3_right_torque$ name=mec_brk_Axle3_right_torque prio=1 dataSetName=std dataClassType=initIO dataClassName=initIO unit='Nm' description='Torque Brake 3 right Wheel': interface_IO.mec_brk_Axle3_right_torque_0 [-]"; p63 "Acceleration Brake 4 (init) export=$sw_mec_brk_Axle4_angAcc$ name=mec_brk_Axle4_angAcc prio=1 dataSetName=std dataClassType=initIO dataClassName=initIO unit='rad/s^2' description='Acceleration Brake 4': interface_IO.mec_brk_Axle4_angAcc_0 [-]"; p64 "Angle Brake 4 (init) export=$sw_mec_brk_Axle4_angPos$ name=mec_brk_Axle4_angPos prio=1 dataSetName=std dataClassType=initIO dataClassName=initIO unit='rad' description='Angle Brake 4': interface_IO.mec_brk_Axle4_angPos_0 [-]"; p65 "Velocity Brake 4 (init) export=$sw_mec_brk_Axle4_angVel$ name=mec_brk_Axle4_angVel prio=1 dataSetName=std dataClassType=initIO dataClassName=initIO unit='rad/s' description='Velocity Brake 4': interface_IO.mec_brk_Axle4_angVel_0 [-]"; p66 "Acceleration Brake 4 left Wheel (init) export=$sw_mec_brk_Axle4_left_angAcc$ name=mec_brk_Axle4_left_angAcc prio=1 dataSetName=std dataClassType=initIO dataClassName=initIO unit='rad/s^2' description='Acceleration Brake 4 left Wheel': interface_IO.mec_brk_Axle4_left_angAcc_0 [-]"; p67 "Angle Brake 4 left Wheel (init) export=$sw_mec_brk_Axle4_left_angPos$ name=mec_brk_Axle4_left_angPos prio=1 dataSetName=std dataClassType=initIO dataClassName=initIO unit='rad' description='Angle Brake 4 left Wheel': interface_IO.mec_brk_Axle4_left_angPos_0 [-]"; p68 "Velocity Brake 4 left Wheel (init) export=$sw_mec_brk_Axle4_left_angVel$ name=mec_brk_Axle4_left_angVel prio=1 dataSetName=std dataClassType=initIO dataClassName=initIO unit='rad/s' description='Velocity Brake 4 left Wheel': interface_IO.mec_brk_Axle4_left_angVel_0 [-]"; p69 "Torque Brake 4 left Wheel (init) export=$sw_mec_brk_Axle4_left_torque$ name=mec_brk_Axle4_left_torque prio=1 dataSetName=std dataClassType=initIO dataClassName=initIO unit='Nm' description='Torque Brake 4 left Wheel': interface_IO.mec_brk_Axle4_left_torque_0 [-]"; p70 "Acceleration Brake 4 right Wheel (init) export=$sw_mec_brk_Axle4_right_angAcc$ name=mec_brk_Axle4_right_angAcc prio=1 dataSetName=std dataClassType=initIO dataClassName=initIO unit='rad/s^2' description='Acceleration Brake 4 right Wheel': interface_IO.mec_brk_Axle4_right_angAcc_0 [-]"; p71 "Angle Brake 4 right Wheel (init) export=$sw_mec_brk_Axle4_right_angPos$ name=mec_brk_Axle4_right_angPos prio=1 dataSetName=std dataClassType=initIO dataClassName=initIO unit='rad' description='Angle Brake 4 right Wheel': interface_IO.mec_brk_Axle4_right_angPos_0 [-]"; p72 "Velocity Brake 4 right Wheel (init) export=$sw_mec_brk_Axle4_right_angVel$ name=mec_brk_Axle4_right_angVel prio=1 dataSetName=std dataClassType=initIO dataClassName=initIO unit='rad/s' description='Velocity Brake 4 right Wheel': interface_IO.mec_brk_Axle4_right_angVel_0 [-]"; p73 "Torque Brake 4 right Wheel (init) export=$sw_mec_brk_Axle4_right_torque$ name=mec_brk_Axle4_right_torque prio=1 dataSetName=std dataClassType=initIO dataClassName=initIO unit='Nm' description='Torque Brake 4 right Wheel': interface_IO.mec_brk_Axle4_right_torque_0 [-]"; p74 "Acceleration Trailer Brake 1 (init) export=$sw_mec_brk_TrailerAxle1_angAcc$ name=mec_brk_TrailerAxle1_angAcc prio=1 dataSetName=std dataClassType=initIO dataClassName=initIO unit='rad/s^2' description='Acceleration Trailer Brake 1': interface_IO.mec_brk_TrailerAxle1_angAcc_0 [-]"; p75 "Angle Trailer Brake 1 (init) export=$sw_mec_brk_TrailerAxle1_angPos$ name=mec_brk_TrailerAxle1_angPos prio=1 dataSetName=std dataClassType=initIO dataClassName=initIO unit='rad' description='Angle Trailer Brake 1': interface_IO.mec_brk_TrailerAxle1_angPos_0 [-]"; p76 "Velocity Trailer Brake 1 (init) export=$sw_mec_brk_TrailerAxle1_angVel$ name=mec_brk_TrailerAxle1_angVel prio=1 dataSetName=std dataClassType=initIO dataClassName=initIO unit='rad/s' description='Velocity Trailer Brake 1': interface_IO.mec_brk_TrailerAxle1_angVel_0 [-]"; p77 "Acceleration Trailer Brake 1 left Wheel (init) export=$sw_mec_brk_TrailerAxle1_left_angAcc$ name=mec_brk_TrailerAxle1_left_angAcc prio=1 dataSetName=std dataClassType=initIO dataClassName=initIO unit='rad/s^2' description='Acceleration Trailer Brake 1 left Wheel': interface_IO.mec_brk_TrailerAxle1_left_angAcc_0 [-]"; p78 "Angle Trailer Brake 1 left Wheel (init) export=$sw_mec_brk_TrailerAxle1_left_angPos$ name=mec_brk_TrailerAxle1_left_angPos prio=1 dataSetName=std dataClassType=initIO dataClassName=initIO unit='rad' description='Angle Trailer Brake 1 left Wheel': interface_IO.mec_brk_TrailerAxle1_left_angPos_0 [-]"; p79 "Velocity Trailer Brake 1 left Wheel (init) export=$sw_mec_brk_TrailerAxle1_left_angVel$ name=mec_brk_TrailerAxle1_left_angVel prio=1 dataSetName=std dataClassType=initIO dataClassName=initIO unit='rad/s' description='Velocity Trailer Brake 1 left Wheel': interface_IO.mec_brk_TrailerAxle1_left_angVel_0 [-]"; p80 "Torque Trailer Brake 1 left Wheel (init) export=$sw_mec_brk_TrailerAxle1_left_torque$ name=mec_brk_TrailerAxle1_left_torque prio=1 dataSetName=std dataClassType=initIO dataClassName=initIO unit='Nm' description='Torque Trailer Brake 1 left Wheel': interface_IO.mec_brk_TrailerAxle1_left_torque_0 [-]"; p81 "Acceleration Trailer Brake 1 right Wheel (init) export=$sw_mec_brk_TrailerAxle1_right_angAcc$ name=mec_brk_TrailerAxle1_right_angAcc prio=1 dataSetName=std dataClassType=initIO dataClassName=initIO unit='rad/s^2' description='Acceleration Trailer Brake 1 right Wheel': interface_IO.mec_brk_TrailerAxle1_right_angAcc_0 [-]"; p82 "Angle Trailer Brake 1 right Wheel (init) export=$sw_mec_brk_TrailerAxle1_right_angPos$ name=mec_brk_TrailerAxle1_right_angPos prio=1 dataSetName=std dataClassType=initIO dataClassName=initIO unit='rad' description='Angle Trailer Brake 1 right Wheel': interface_IO.mec_brk_TrailerAxle1_right_angPos_0 [-]"; p83 "Velocity Trailer Brake 1 right Wheel (init) export=$sw_mec_brk_TrailerAxle1_right_angVel$ name=mec_brk_TrailerAxle1_right_angVel prio=1 dataSetName=std dataClassType=initIO dataClassName=initIO unit='rad/s' description='Velocity Trailer Brake 1 right Wheel': interface_IO.mec_brk_TrailerAxle1_right_angVel_0 [-]"; p84 "Torque Trailer Brake 1 right Wheel (init) export=$sw_mec_brk_TrailerAxle1_right_torque$ name=mec_brk_TrailerAxle1_right_torque prio=1 dataSetName=std dataClassType=initIO dataClassName=initIO unit='Nm' description='Torque Trailer Brake 1 right Wheel': interface_IO.mec_brk_TrailerAxle1_right_torque_0 [-]"; p85 "Acceleration Trailer Brake 2 (init) export=$sw_mec_brk_TrailerAxle2_angAcc$ name=mec_brk_TrailerAxle2_angAcc prio=1 dataSetName=std dataClassType=initIO dataClassName=initIO unit='rad/s^2' description='Acceleration Trailer Brake 2': interface_IO.mec_brk_TrailerAxle2_angAcc_0 [-]"; p86 "Angle Trailer Brake 2 (init) export=$sw_mec_brk_TrailerAxle2_angPos$ name=mec_brk_TrailerAxle2_angPos prio=1 dataSetName=std dataClassType=initIO dataClassName=initIO unit='rad' description='Angle Trailer Brake 2': interface_IO.mec_brk_TrailerAxle2_angPos_0 [-]"; p87 "Velocity Trailer Brake 2 (init) export=$sw_mec_brk_TrailerAxle2_angVel$ name=mec_brk_TrailerAxle2_angVel prio=1 dataSetName=std dataClassType=initIO dataClassName=initIO unit='rad/s' description='Velocity Trailer Brake 2': interface_IO.mec_brk_TrailerAxle2_angVel_0 [-]"; p88 "Acceleration Trailer Brake 2 left Wheel (init) export=$sw_mec_brk_TrailerAxle2_left_angAcc$ name=mec_brk_TrailerAxle2_left_angAcc prio=1 dataSetName=std dataClassType=initIO dataClassName=initIO unit='rad/s^2' description='Acceleration Trailer Brake 2 left Wheel': interface_IO.mec_brk_TrailerAxle2_left_angAcc_0 [-]"; p89 "Angle Trailer Brake 2 left Wheel (init) export=$sw_mec_brk_TrailerAxle2_left_angPos$ name=mec_brk_TrailerAxle2_left_angPos prio=1 dataSetName=std dataClassType=initIO dataClassName=initIO unit='rad' description='Angle Trailer Brake 2 left Wheel': interface_IO.mec_brk_TrailerAxle2_left_angPos_0 [-]"; p90 "Velocity Trailer Brake 2 left Wheel (init) export=$sw_mec_brk_TrailerAxle2_left_angVel$ name=mec_brk_TrailerAxle2_left_angVel prio=1 dataSetName=std dataClassType=initIO dataClassName=initIO unit='rad/s' description='Velocity Trailer Brake 2 left Wheel': interface_IO.mec_brk_TrailerAxle2_left_angVel_0 [-]"; p91 "Torque Trailer Brake 2 left Wheel (init) export=$sw_mec_brk_TrailerAxle2_left_torque$ name=mec_brk_TrailerAxle2_left_torque prio=1 dataSetName=std dataClassType=initIO dataClassName=initIO unit='Nm' description='Torque Trailer Brake 2 left Wheel': interface_IO.mec_brk_TrailerAxle2_left_torque_0 [-]"; p92 "Acceleration Trailer Brake 2 right Wheel (init) export=$sw_mec_brk_TrailerAxle2_right_angAcc$ name=mec_brk_TrailerAxle2_right_angAcc prio=1 dataSetName=std dataClassType=initIO dataClassName=initIO unit='rad/s^2' description='Acceleration Trailer Brake 2 right Wheel': interface_IO.mec_brk_TrailerAxle2_right_angAcc_0 [-]"; p93 "Angle Trailer Brake 2 right Wheel (init) export=$sw_mec_brk_TrailerAxle2_right_angPos$ name=mec_brk_TrailerAxle2_right_angPos prio=1 dataSetName=std dataClassType=initIO dataClassName=initIO unit='rad' description='Angle Trailer Brake 2 right Wheel': interface_IO.mec_brk_TrailerAxle2_right_angPos_0 [-]"; p94 "Velocity Trailer Brake 2 right Wheel (init) export=$sw_mec_brk_TrailerAxle2_right_angVel$ name=mec_brk_TrailerAxle2_right_angVel prio=1 dataSetName=std dataClassType=initIO dataClassName=initIO unit='rad/s' description='Velocity Trailer Brake 2 right Wheel': interface_IO.mec_brk_TrailerAxle2_right_angVel_0 [-]"; p95 "Torque Trailer Brake 2 right Wheel (init) export=$sw_mec_brk_TrailerAxle2_right_torque$ name=mec_brk_TrailerAxle2_right_torque prio=1 dataSetName=std dataClassType=initIO dataClassName=initIO unit='Nm' description='Torque Trailer Brake 2 right Wheel': interface_IO.mec_brk_TrailerAxle2_right_torque_0 [-]"; p96 "Acceleration Trailer Brake 3 (init) export=$sw_mec_brk_TrailerAxle3_angAcc$ name=mec_brk_TrailerAxle3_angAcc prio=1 dataSetName=std dataClassType=initIO dataClassName=initIO unit='rad/s^2' description='Acceleration Trailer Brake 3': interface_IO.mec_brk_TrailerAxle3_angAcc_0 [-]"; p97 "Angle Trailer Brake 3 (init) export=$sw_mec_brk_TrailerAxle3_angPos$ name=mec_brk_TrailerAxle3_angPos prio=1 dataSetName=std dataClassType=initIO dataClassName=initIO unit='rad' description='Angle Trailer Brake 3': interface_IO.mec_brk_TrailerAxle3_angPos_0 [-]"; p98 "Velocity Trailer Brake 3 (init) export=$sw_mec_brk_TrailerAxle3_angVel$ name=mec_brk_TrailerAxle3_angVel prio=1 dataSetName=std dataClassType=initIO dataClassName=initIO unit='rad/s' description='Velocity Trailer Brake 3': interface_IO.mec_brk_TrailerAxle3_angVel_0 [-]"; p99 "Acceleration Trailer Brake 3 left Wheel (init) export=$sw_mec_brk_TrailerAxle3_left_angAcc$ name=mec_brk_TrailerAxle3_left_angAcc prio=1 dataSetName=std dataClassType=initIO dataClassName=initIO unit='rad/s^2' description='Acceleration Trailer Brake 3 left Wheel': interface_IO.mec_brk_TrailerAxle3_left_angAcc_0 [-]"; p100 "Angle Trailer Brake 3 left Wheel (init) export=$sw_mec_brk_TrailerAxle3_left_angPos$ name=mec_brk_TrailerAxle3_left_angPos prio=1 dataSetName=std dataClassType=initIO dataClassName=initIO unit='rad' description='Angle Trailer Brake 3 left Wheel': interface_IO.mec_brk_TrailerAxle3_left_angPos_0 [-]"; p101 "Velocity Trailer Brake 3 left Wheel (init) export=$sw_mec_brk_TrailerAxle3_left_angVel$ name=mec_brk_TrailerAxle3_left_angVel prio=1 dataSetName=std dataClassType=initIO dataClassName=initIO unit='rad/s' description='Velocity Trailer Brake 3 left Wheel': interface_IO.mec_brk_TrailerAxle3_left_angVel_0 [-]"; p102 "Torque Trailer Brake 3 left Wheel (init) export=$sw_mec_brk_TrailerAxle3_left_torque$ name=mec_brk_TrailerAxle3_left_torque prio=1 dataSetName=std dataClassType=initIO dataClassName=initIO unit='Nm' description='Torque Trailer Brake 3  left Wheel': interface_IO.mec_brk_TrailerAxle3_left_torque_0 [-]"; p103 "Acceleration Trailer Brake 3 right Wheel (init) export=$sw_mec_brk_TrailerAxle3_right_angAcc$ name=mec_brk_TrailerAxle3_right_angAcc prio=1 dataSetName=std dataClassType=initIO dataClassName=initIO unit='rad/s^2' description='Acceleration Trailer Brake 3 right Wheel': interface_IO.mec_brk_TrailerAxle3_right_angAcc_0 [-]"; p104 "Angle Trailer Brake 3 right Wheel (init) export=$sw_mec_brk_TrailerAxle3_right_angPos$ name=mec_brk_TrailerAxle3_right_angPos prio=1 dataSetName=std dataClassType=initIO dataClassName=initIO unit='rad' description='Angle Trailer Brake 3 right Wheel': interface_IO.mec_brk_TrailerAxle3_right_angPos_0 [-]"; p105 "Velocity Trailer Brake 3 right Wheel (init) export=$sw_mec_brk_TrailerAxle3_right_angVel$ name=mec_brk_TrailerAxle3_right_angVel prio=1 dataSetName=std dataClassType=initIO dataClassName=initIO unit='rad/s' description='Velocity Trailer Brake 3 right Wheel': interface_IO.mec_brk_TrailerAxle3_right_angVel_0 [-]"; p106 "Torque Trailer Brake 3 right Wheel (init) export=$sw_mec_brk_TrailerAxle3_right_torque$ name=mec_brk_TrailerAxle3_right_torque prio=1 dataSetName=std dataClassType=initIO dataClassName=initIO unit='Nm' description='Torque Trailer Brake 3  right Wheel': interface_IO.mec_brk_TrailerAxle3_right_torque_0 [-]"; p107 "Torque Engine Crankshaft (init) export=$sw_mec_eng_CrankMean_torque$ name=mec_eng_CrankMean_torque prio=1 dataSetName=std dataClassType=initIO dataClassName=initIO unit='Nm' description='Torque Engine Crankshaft': interface_IO.mec_eng_CrankMean_torque_0 [-]"; p108 "Acceleration Retarder (init) export=$sw_mec_ret_Retarder_angAcc$ name=mec_ret_Retarder_angAcc prio=1 dataSetName=std dataClassType=initIO dataClassName=initIO unit='rad/s^2' description='Acceleration Retarder': interface_IO.mec_ret_Retarder_angAcc_0 [-]"; p109 "Angle Retarder (init) export=$sw_mec_ret_Retarder_angPos$ name=mec_ret_Retarder_angPos prio=1 dataSetName=std dataClassType=initIO dataClassName=initIO unit='rad' description='Angle Retarder': interface_IO.mec_ret_Retarder_angPos_0 [-]"; p110 "Velocity  Retarder (init) export=$sw_mec_ret_Retarder_angVel$ name=mec_ret_Retarder_angVel prio=1 dataSetName=std dataClassType=initIO dataClassName=initIO unit='rad/s' description='Velocity Retarder': interface_IO.mec_ret_Retarder_angVel_0 [-]"; p111 "Torque Retarder (init) export=$sw_mec_ret_Retarder_torque$ name=mec_ret_Retarder_torque prio=1 dataSetName=std dataClassType=initIO dataClassName=initIO unit='Nm' description='Torque Retarder': interface_IO.mec_ret_Retarder_torque_0 [-]"; p112 "Transmission sensor road inclination (init) export=$sw_mec_tx_inclRoadSns$ name=mec_tx_inclRoadSns prio=1 dataSetName=std dataClassType=initIO dataClassName=initIO unit='deg' description='Transmission sensor road inclination': interface_IO.mec_tx_inclRoadSns_0 [-]"; p113 "Speed sensor Transmission output (init) export=$sw_mec_tx_nGbOutD3Sns$ name=mec_tx_nGbOutD3Sns prio=1 dataSetName=std dataClassType=initIO dataClassName=initIO unit='rpm' description='Speed sensor Transmission output': interface_IO.mec_tx_nGbOutD3Sns_0 [-]"; p114 "Speed sensor Transmission output (init) export=$sw_mec_tx_nGbOutDzAwSns$ name=mec_tx_nGbOutDzAwSns prio=1 dataSetName=std dataClassType=initIO dataClassName=initIO unit='rpm' description='Speed sensor Transmission output': interface_IO.mec_tx_nGbOutDzAwSns_0 [-]"; p115 "Speed sensor Transmission output (init) export=$sw_mec_tx_nGbOutDzSfSns$ name=mec_tx_nGbOutDzSfSns prio=1 dataSetName=std dataClassType=initIO dataClassName=initIO unit='rpm' description='Speed sensor Transmission output': interface_IO.mec_tx_nGbOutDzSfSns_0 [-]"; p116 "Speed sensor Transmission output (init) export=$sw_mec_tx_nGbOutDzTuAwSns$ name=mec_tx_nGbOutDzTuAwSns prio=1 dataSetName=std dataClassType=initIO dataClassName=initIO unit='rpm' description='Speed sensor Transmission output': interface_IO.mec_tx_nGbOutDzTuAwSns_0 [-]"; p117 "Speed sensor Transmission output (init) export=$sw_mec_tx_nGbOutSns$ name=mec_tx_nGbOutSns prio=1 dataSetName=std dataClassType=initIO dataClassName=initIO unit='rpm' description='Speed sensor Transmission output': interface_IO.mec_tx_nGbOutSns_0 [-]"; p118 "Axle Load 1 (init) export=$sw_mec_veh_AxleLoad1$ name=mec_veh_AxleLoad1 prio=1 dataSetName=std dataClassType=initIO dataClassName=initIO unit='m' description='Vehicle position': interface_IO.mec_veh_AxleLoad1_0 [-]"; p119 "Axle Load 2 (init) export=$sw_mec_veh_AxleLoad2$ name=mec_veh_AxleLoad2 prio=1 dataSetName=std dataClassType=initIO dataClassName=initIO unit='m' description='Vehicle position': interface_IO.mec_veh_AxleLoad2_0 [-]"; p120 "Axle Load 3 (init) export=$sw_mec_veh_AxleLoad3$ name=mec_veh_AxleLoad3 prio=1 dataSetName=std dataClassType=initIO dataClassName=initIO unit='m' description='Vehicle position': interface_IO.mec_veh_AxleLoad3_0 [-]"; p121 "Axle Load 4 (init) export=$sw_mec_veh_AxleLoad4$ name=mec_veh_AxleLoad4 prio=1 dataSetName=std dataClassType=initIO dataClassName=initIO unit='m' description='Vehicle position': interface_IO.mec_veh_AxleLoad4_0 [-]"; p122 "Roll Coefficient Overall (init) export=$sw_mec_veh_fRollCoeffOverall$ name=mec_veh_fRollCoeffOverall prio=1 dataSetName=std dataClassType=initIO dataClassName=initIO unit='m' description='Vehicle position': interface_IO.mec_veh_fRollCoeffOverall_0 [-]"; p123 "Force Generic Vehicle Loss (init) export=$sw_mec_veh_GenericLoss_force$ name=mec_veh_GenericLoss_force prio=1 dataSetName=std dataClassType=initIO dataClassName=initIO unit='N' description='Force Generic Vehicle Loss': interface_IO.mec_veh_GenericLoss_force_0 [-]"; p124 "Acceleration Generic Vehicle Loss (init) export=$sw_mec_veh_GenericLoss_transAcc$ name=mec_veh_GenericLoss_transAcc prio=1 dataSetName=std dataClassType=initIO dataClassName=initIO unit='m/s^2' description='Acceleration Generic Vehicle Loss': interface_IO.mec_veh_GenericLoss_transAcc_0 [-]"; p125 "Position Generic Vehicle Loss (init) export=$sw_mec_veh_GenericLoss_transPos$ name=mec_veh_GenericLoss_transPos prio=1 dataSetName=std dataClassType=initIO dataClassName=initIO unit='m' description='Position Generic Vehicle Loss': interface_IO.mec_veh_GenericLoss_transPos_0 [-]"; p126 "Velocity Generic Vehicle Loss (init) export=$sw_mec_veh_GenericLoss_transVel$ name=mec_veh_GenericLoss_transVel prio=1 dataSetName=std dataClassType=initIO dataClassName=initIO unit='m/s' description='Veloctiy Generic Vehicle Loss': interface_IO.mec_veh_GenericLoss_transVel_0 [-]"; p127 "Vehicle mass (init) export=$sw_mec_veh_massVehicle$ name=mec_veh_massVehicle prio=1 dataSetName=std dataClassType=initIO dataClassName=initIO unit='kg' description='Vehicle mass': interface_IO.mec_veh_massVehicle_0 [-]"; p128 "Payload Mass (init) export=$sw_mec_veh_Payload$ name=mec_veh_Payload prio=1 dataSetName=std dataClassType=initIO dataClassName=initIO unit='m' description='Vehicle position': interface_IO.mec_veh_Payload_0 [-]"; p129 "Total GroComb Weight(init) export=$sw_mec_veh_TotalGroCombWeight$ name=mec_veh_TotalGroCombWeight prio=1 dataSetName=std dataClassType=initIO dataClassName=initIO unit='m' description='Vehicle position': interface_IO.mec_veh_TotalGroCombWeight_0 [-]"; p130 "TrailerAxle Load 1 (init) export=$sw_mec_veh_TrailerAxleLoad1$ name=mec_veh_TrailerAxleLoad1 prio=1 dataSetName=std dataClassType=initIO dataClassName=initIO unit='m' description='Vehicle position': interface_IO.mec_veh_TrailerAxleLoad1_0 [-]"; p131 "TrailerAxle Load 2 (init) export=$sw_mec_veh_TrailerAxleLoad2$ name=mec_veh_TrailerAxleLoad2 prio=1 dataSetName=std dataClassType=initIO dataClassName=initIO unit='m' description='Vehicle position': interface_IO.mec_veh_TrailerAxleLoad2_0 [-]"; p132 "TrailerAxle Load 3 (init) export=$sw_mec_veh_TrailerAxleLoad3$ name=mec_veh_TrailerAxleLoad3 prio=1 dataSetName=std dataClassType=initIO dataClassName=initIO unit='m' description='Vehicle position': interface_IO.mec_veh_TrailerAxleLoad3_0 [-]"; p133 "Vehicle acceleration (init) export=$sw_mec_veh_transAcc$ name=mec_veh_transAcc prio=1 dataSetName=std dataClassType=initIO dataClassName=initIO unit='m/s^2' description='Vehicle acceleration': interface_IO.mec_veh_transAcc_0 [-]"; p134 "Vehicle position (init) export=$sw_mec_veh_transPos$ name=mec_veh_transPos prio=1 dataSetName=std dataClassType=initIO dataClassName=initIO unit='m' description='Vehicle position': interface_IO.mec_veh_transPos_0 [-]"; p135 "Vehicle speed (real speed of vehicle) (init) export=$sw_mec_veh_transVel$ name=mec_veh_transVel prio=1 dataSetName=std dataClassType=initIO dataClassName=initIO unit='m/s' description='Vehicle speed': interface_IO.mec_veh_transVel_0 [-]"; p136 "Vehicle Speed (physical reference value) (init) export=$sw_mec_veh_VehVelReferenceCool_velocity$ name=mec_veh_VehVelReferenceCool_velocity prio=1 dataSetName=std dataClassType=initIO dataClassName=initIO unit='m/s^2' description='Vehicle Speed (physical reference value)': interface_IO.mec_veh_VehVelReferenceCool_velocity_0 [-]"; p137 "Vehicle Speed (physical reference value) (init) export=$sw_mec_veh_VehVelReferenceUhood_velocity$ name=mec_veh_VehVelReferenceUhood_velocity prio=1 dataSetName=std dataClassType=initIO dataClassName=initIO unit='m/s^2' description='Vehicle Speed (physical reference value)': interface_IO.mec_veh_VehVelReferenceUhood_velocity_0 [-]"; p138 "Acceleration Generic Wheel Loss (init) export=$sw_mec_wheel_GenericLoss_angAcc$ name=mec_wheel_GenericLoss_angAcc prio=1 dataSetName=std dataClassType=initIO dataClassName=initIO unit='rad/s^2' description='Acceleration Generic Wheel Loss': interface_IO.mec_wheel_GenericLoss_angAcc_0 [-]"; p139 "Angle Generic Wheel Loss (init) export=$sw_mec_wheel_GenericLoss_angPos$ name=mec_wheel_GenericLoss_angPos prio=1 dataSetName=std dataClassType=initIO dataClassName=initIO unit='rad' description='Angle Generic Wheel Loss': interface_IO.mec_wheel_GenericLoss_angPos_0 [-]"; p140 "Velocity Generic Wheel Loss (init) export=$sw_mec_wheel_GenericLoss_angVel$ name=mec_wheel_GenericLoss_angVel prio=1 dataSetName=std dataClassType=initIO dataClassName=initIO unit='rad/s' description='Velocity Generic Wheel Loss': interface_IO.mec_wheel_GenericLoss_angVel_0 [-]"; p141 "Torque Generic Wheel Loss (init) export=$sw_mec_wheel_GenericLoss_torque$ name=mec_wheel_GenericLoss_torque prio=1 dataSetName=std dataClassType=initIO dataClassName=initIO unit='Nm' description='Torque Generic Wheel Loss': interface_IO.mec_wheel_GenericLoss_torque_0 [-]"; p142 "[rpm] export=true prio=1 name=mec_brk_Axle1_omBrk_info dataSetName=std dataClassType=initIO dataClassName=initIO unit='rpm' description='-': mec_brk_Axle1_omBrk_info_0 [-]"; p143 "[rpm] export=true name=mec_brk_Axle1_omIn_info prio=1 dataSetName=std dataClassType=initIO dataClassName=initIO unit='rpm' description='-': mec_brk_Axle1_omIn_info_0 [-]"; p144 "[Nm] export=true prio=1 name=mec_brk_Axle1_TiBrk_info dataSetName=std dataClassType=initIO dataClassName=initIO unit='Nm' description='-': mec_brk_Axle1_TiBrk_info_0 [-]"; p145 "[Nm] export=true prio=1 name=mec_brk_Axle1_TiLoss_info dataSetName=std dataClassType=initIO dataClassName=initIO unit='Nm' description='-': mec_brk_Axle1_TiLoss_info_0 [-]"; p146 "[Nm] export=true name=mec_brk_Axle1_TIn_info prio=1 dataSetName=std dataClassType=initIO dataClassName=initIO unit='Nm' description='-': mec_brk_Axle1_TIn_info_0 [-]"; p147 "[rpm] export=true name=mec_brk_Axle2_omIn_info prio=1 dataSetName=std dataClassType=initIO dataClassName=initIO unit='rpm' description='-': mec_brk_Axle2_omIn_info_0 [-]"; p148 "[Nm] export=true prio=1 name=mec_brk_Axle2_TiBrk_info dataSetName=std dataClassType=initIO dataClassName=initIO unit='Nm' description='-': mec_brk_Axle2_TiBrk_info_0 [-]"; p149 "[Nm] export=true prio=1 name=mec_brk_Axle2_TiLoss_info dataSetName=std dataClassType=initIO dataClassName=initIO unit='Nm' description='-': mec_brk_Axle2_TiLoss_info_0 [-]"; p150 "[Nm] export=true name=mec_brk_Axle2_TIn_info prio=1 dataSetName=std dataClassType=initIO dataClassName=initIO unit='Nm' description='-': mec_brk_Axle2_TIn_info_0 [-]"; p151 "[rpm] export=true name=mec_brk_Axle3_omIn_info prio=1 dataSetName=std dataClassType=initIO dataClassName=initIO unit='rpm' description='-': mec_brk_Axle3_omIn_info_0 [-]"; p152 "[Nm] export=true prio=1 name=mec_brk_Axle3_TiBrk_info dataSetName=std dataClassType=initIO dataClassName=initIO unit='Nm' description='-': mec_brk_Axle3_TiBrk_info_0 [-]"; p153 "[Nm] export=true prio=1 name=mec_brk_Axle3_TiLoss_info dataSetName=std dataClassType=initIO dataClassName=initIO unit='Nm' description='-': mec_brk_Axle3_TiLoss_info_0 [-]"; p154 "[Nm] export=true name=mec_brk_Axle3_TIn_info prio=1 dataSetName=std dataClassType=initIO dataClassName=initIO unit='Nm' description='-': mec_brk_Axle3_TIn_info_0 [-]"; p155 "[rpm] export=true name=mec_brk_Axle4_omIn_info prio=1 dataSetName=std dataClassType=initIO dataClassName=initIO unit='rpm' description='-': mec_brk_Axle4_omIn_info_0 [-]"; p156 "[Nm] export=true prio=1 name=mec_brk_Axle4_TiBrk_info dataSetName=std dataClassType=initIO dataClassName=initIO unit='Nm' description='-': mec_brk_Axle4_TiBrk_info_0 [-]"; p157 "[Nm] export=true prio=1 name=mec_brk_Axle4_TiLoss_info dataSetName=std dataClassType=initIO dataClassName=initIO unit='Nm' description='-': mec_brk_Axle4_TiLoss_info_0 [-]"; p158 "[Nm] export=true name=mec_brk_Axle4_TIn_info prio=1 dataSetName=std dataClassType=initIO dataClassName=initIO unit='Nm' description='-': mec_brk_Axle4_TIn_info_0 [-]"; p159 "[rpm] export=true name=mec_brk_TrailerAxle1_omIn_info prio=1 dataSetName=std dataClassType=initIO dataClassName=initIO unit='rpm' description='-': mec_brk_TrailerAxle1_omIn_info_0 [-]"; p160 "[Nm] export=true prio=1 name=mec_brk_TrailerAxle1_TiBrk_info dataSetName=std dataClassType=initIO dataClassName=initIO unit='Nm' description='-': mec_brk_TrailerAxle1_TiBrk_info_0 [-]"; p161 "[Nm] export=true prio=1 name=mec_brk_TrailerAxle1_TiLoss_info dataSetName=std dataClassType=initIO dataClassName=initIO unit='Nm' description='-': mec_brk_TrailerAxle1_TiLoss_info_0 [-]"; p162 "[Nm] export=true name=mec_brk_TrailerAxle1_TIn_info prio=1 dataSetName=std dataClassType=initIO dataClassName=initIO unit='Nm' description='-': mec_brk_TrailerAxle1_TIn_info_0 [-]"; p163 "[rpm] export=true name=mec_brk_TrailerAxle2_omIn_info prio=1 dataSetName=std dataClassType=initIO dataClassName=initIO unit='rpm' description='-': mec_brk_TrailerAxle2_omIn_info_0 [-]"; p164 "[Nm] export=true prio=1 name=mec_brk_TrailerAxle2_TiBrk_info dataSetName=std dataClassType=initIO dataClassName=initIO unit='Nm' description='-': mec_brk_TrailerAxle2_TiBrk_info_0 [-]"; p165 "[Nm] export=true prio=1 name=mec_brk_TrailerAxle2_TiLoss_info dataSetName=std dataClassType=initIO dataClassName=initIO unit='Nm' description='-': mec_brk_TrailerAxle2_TiLoss_info_0 [-]"; p166 "[Nm] export=true name=mec_brk_TrailerAxle2_TIn_info prio=1 dataSetName=std dataClassType=initIO dataClassName=initIO unit='Nm' description='-': mec_brk_TrailerAxle2_TIn_info_0 [-]"; p167 "[rpm] export=true name=mec_brk_TrailerAxle3_omIn_info prio=1 dataSetName=std dataClassType=initIO dataClassName=initIO unit='rpm' description='-': mec_brk_TrailerAxle3_omIn_info_0 [-]"; p168 "[Nm] export=true prio=1 name=mec_brk_TrailerAxle3_TiBrk_info dataSetName=std dataClassType=initIO dataClassName=initIO unit='Nm' description='-': mec_brk_TrailerAxle3_TiBrk_info_0 [-]"; p169 "[Nm] export=true prio=1 name=mec_brk_TrailerAxle3_TiLoss_info dataSetName=std dataClassType=initIO dataClassName=initIO unit='Nm' description='-': mec_brk_TrailerAxle3_TiLoss_info_0 [-]"; p170 "[Nm] export=true name=mec_brk_TrailerAxle3_TIn_info prio=1 dataSetName=std dataClassType=initIO dataClassName=initIO unit='Nm' description='-': mec_brk_TrailerAxle3_TIn_info_0 [-]"; p171 "[Nm] export=true prio=1 name=mec_brk_TrailerWheel1_TiLossRollRes_info dataSetName=std dataClassType=initIO dataClassName=initIO unit='Nm' description='-': mec_brk_TrailerWheel1_TiLossRollRes_info_0 [-]"; p172 "[Nm] export=true prio=1 name=mec_brk_TrailerWheel2_TiLossRollRes_info dataSetName=std dataClassType=initIO dataClassName=initIO unit='Nm' description='-': mec_brk_TrailerWheel2_TiLossRollRes_info_0 [-]"; p173 "[Nm] export=true prio=1 name=mec_brk_TrailerWheel3_TiLossRollRes_info dataSetName=std dataClassType=initIO dataClassName=initIO unit='Nm' description='-': mec_brk_TrailerWheel3_TiLossRollRes_info_0 [-]"; p174 "[Nm] export=true prio=1 name=mec_brk_Wheel1_TiLossRollRes_info dataSetName=std dataClassType=initIO dataClassName=initIO unit='Nm' description='-': mec_brk_Wheel1_TiLossRollRes_info_0 [-]"; p175 "[Nm] export=true prio=1 name=mec_brk_Wheel2_TiLossRollRes_info dataSetName=std dataClassType=initIO dataClassName=initIO unit='Nm' description='-': mec_brk_Wheel2_TiLossRollRes_info_0 [-]"; p176 "[Nm] export=true prio=1 name=mec_brk_Wheel3_TiLossRollRes_info dataSetName=std dataClassType=initIO dataClassName=initIO unit='Nm' description='-': mec_brk_Wheel3_TiLossRollRes_info_0 [-]"; p177 "[Nm] export=true prio=1 name=mec_brk_Wheel4_TiLossRollRes_info dataSetName=std dataClassType=initIO dataClassName=initIO unit='Nm' description='-': mec_brk_Wheel4_TiLossRollRes_info_0 [-]"; p178 "[Nm] export=true name=mec_ret_T_info prio=1 dataSetName=std dataClassType=initIO dataClassName=initIO unit='Nm' description='-': mec_ret_T_info_0 [-]"; p179 "[rpm] export=true prio=1 name=mec_sht_omShtF_info dataSetName=std dataClassType=initIO dataClassName=initIO unit='rpm' description='-': mec_sht_omShtF_info_0 [-]"; p180 "[rpm] export=true prio=1 name=mec_sht_omShtR_info dataSetName=std dataClassType=initIO dataClassName=initIO unit='rpm' description='-': mec_sht_omShtR_info_0 [-]"; p181 "[rpm] export=true prio=1 name=mec_sht_TiLossShtF_info dataSetName=std dataClassType=initIO dataClassName=initIO unit='Nm' description='-': mec_sht_TiLossShtF_info_0 [-]"; p182 "[rpm] export=true prio=1 name=mec_sht_TiLossShtR_info dataSetName=std dataClassType=initIO dataClassName=initIO unit='Nm' description='-': mec_sht_TiLossShtR_info_0 [-]"; p183 "[rpm] export=true name=mec_tfc_omOut_info prio=1 dataSetName=std dataClassType=initIO dataClassName=initIO unit='rpm' description='-': mec_tfc_omOut_info_0 [-]"; p184 "[Nm] export=true prio=1 name=mec_tfc_TiLoss_info dataSetName=std dataClassType=initIO dataClassName=initIO unit='Nm' description='-': mec_tfc_TiLoss_info_0 [-]"; p185 "[Nm] export=true prio=1 name=mec_tfc_TOutFront_info dataSetName=std dataClassType=initIO dataClassName=initIO unit='Nm' description='-': mec_tfc_TOutFront_info_0 [-]"; p186 "[Nm] export=true prio=1 name=mec_tfc_TOutRear_info dataSetName=std dataClassType=initIO dataClassName=initIO unit='Nm' description='-': mec_tfc_TOutRear_info_0 [-]"; p187 "[rpm] export=true prio=1 name=mec_veh_domFW_info dataSetName=std dataClassType=initIO dataClassName=initIO unit='rpm' description='-': mec_veh_domFW_info_0 [-]"; p188 "[rad] export=true prio=1 name=mec_veh_dphiFW_info dataSetName=std dataClassType=initIO dataClassName=initIO unit='rad' description='-': mec_veh_dphiFW_info_0 [-]"; p189 "[N] export=true prio=1 name=mec_veh_FiAirDrag_info dataSetName=std dataClassType=initIO dataClassName=initIO unit='N' description='-': mec_veh_FiAirDrag_info_0 [-]"; p190 "[N] export=true prio=1 name=mec_veh_FiGradeRes_info dataSetName=std dataClassType=initIO dataClassName=initIO unit='N' description='-': mec_veh_FiGradeRes_info_0 [-]"; p191 "[N] export=true name=mec_veh_FWheelTraction_info prio=1 dataSetName=std dataClassType=initIO dataClassName=initIO unit='N' description='-': mec_veh_FWheelTraction_info_0 [-]"; p192 "[-] export=true prio=1 name=mec_veh_sFW_info dataSetName=std dataClassType=initIO dataClassName=initIO unit='-' description='-': mec_veh_sFW_info_0 [-]"; p193 "[Nm] export=true prio=1 name=mec_veh_TiFW_info dataSetName=std dataClassType=initIO dataClassName=initIO unit='Nm' description='-': mec_veh_TiFW_info_0 [-]"; p194 "[rpm] export=true prio=1 name=mec_veh_vehConfig_info dataSetName=std dataClassType=initIO dataClassName=initIO unit='rpm' description='-': mec_veh_vehConfig_info_0 [-]"; p195 "[Nm] export=true name=mec_wheel_Axle1_T_info prio=1 dataSetName=std dataClassType=initIO dataClassName=initIO unit='Nm' description='-': mec_wheel_Axle1_T_info_0 [-]"; p196 "[Nm] export=true name=mec_wheel_Axle2_T_info prio=1 dataSetName=std dataClassType=initIO dataClassName=initIO unit='Nm' description='-': mec_wheel_Axle2_T_info_0 [-]"; p197 "[Nm] export=true name=mec_wheel_Axle3_T_info prio=1 dataSetName=std dataClassType=initIO dataClassName=initIO unit='Nm' description='-': mec_wheel_Axle3_T_info_0 [-]"; p198 "[Nm] export=true name=mec_wheel_Axle4_T_info prio=1 dataSetName=std dataClassType=initIO dataClassName=initIO unit='Nm' description='-': mec_wheel_Axle4_T_info_0 [-]"; p199 "[Nm] export=true name=mec_wheel_TrailerAxle1_T_info prio=1 dataSetName=std dataClassType=initIO dataClassName=initIO unit='Nm' description='-': mec_wheel_TrailerAxle1_T_info_0 [-]"; p200 "[Nm] export=true name=mec_wheel_TrailerAxle2_T_info prio=1 dataSetName=std dataClassType=initIO dataClassName=initIO unit='Nm' description='-': mec_wheel_TrailerAxle2_T_info_0 [-]"; p201 "[Nm] export=true name=mec_wheel_TrailerAxle3_T_info prio=1 dataSetName=std dataClassType=initIO dataClassName=initIO unit='Nm' description='-': mec_wheel_TrailerAxle3_T_info_0 [-]"; p202 "Inertia propeller shaft complete [kgm^2] export=true name=JPropShaft_kgm2 prio=1 dataSetName=sht_dummy dataClassType=sht dataClassName=$dataClassNamePropShaft$ unit='kgm^2' description='Inertia Cardanshaft complete': propShaft_front.JPropShaft_kgm2 [kgm²]"; p203 "Inertia propeller shaft complete [kgm^2] export=true name=JPropShaft_kgm2 prio=1 dataSetName=sht_dummy dataClassType=sht dataClassName=$dataClassNamePropShaft$ unit='kgm^2' description='Inertia Cardanshaft complete': propShaft_rear.JPropShaft_kgm2 [kgm²]"; p204 "Ratio Retarder [-] export=true name=iRet prio=1 dataSetName=ret_dummy dataClassType=ret dataClassName=ret unit='-' description='Ratio Retarder': retarder.iRet [-]"; p205 "Inertia Retarder [kgm^2] export=true name=JRet_kgm2 prio=1 dataSetName=ret_dummy dataClassType=ret dataClassName=ret unit='kgm^2' description='Inertia Retarder': retarder.JRet_kgm2 [kgm²]"; p206 "Inertia Retarder drive Gear[kgm^2] export=true name=JRetdrvgear_kgm2 prio=1 dataSetName=ret_dummy dataClassType=ret dataClassName=ret unit='kgm^2' description='Inertia Retarder Drive Gear': retarder.JRetdrvgear_kgm2 [kgm²]"; p207 "Ratio Differential Gear [-] export=true name=iDiff prio=1 dataSetName=axle_dummy dataClassType=axle dataClassName=$dataClassNameAxle$ moduleXmlReference=$moduleXmlReferenceAxle$ unit='-' description='Ratio Differential Gear': trailerAxle1.iDiff [-]"; p208 "Is driven Axle? [-] export=true name=isDriven prio=1 dataSetName=axle_dummy dataClassType=axle dataClassName=$dataClassNameAxle$ moduleXmlReference=$moduleXmlReferenceAxle$ unit='-' description='Is Driven Axle': trailerAxle1.isDriven [-]"; p209 "Is rear Axle? [-] export=true name=isRearAxle prio=1 dataSetName=axle_dummy dataClassType=axle dataClassName=$dataClassNameAxle$ moduleXmlReference=$moduleXmlReferenceAxle$ unit='-' description='Is Rear Axle': trailerAxle1.isRearAxle [-]"; p210 "Inertia Brake Disc  [kgm^2] export=true name=JBrakeDisc_kgm2 prio=1 dataSetName=brk_dummy dataClassType=brk dataClassName=$dataClassNameBrk$ moduleXmlReference=$moduleXmlReferenceBrk$ unit='kgm^2' description='Inertia Brake Disc': trailerAxle1.JBrakeDisc_kgm2 [kgm²]"; p211 "Inertia Hub  [kgm^2] export=true name=JHub_kgm2 prio=1 dataSetName=brk_dummy dataClassType=brk dataClassName=$dataClassNameBrk$ moduleXmlReference=$moduleXmlReferenceBrk$ unit='kgm^2' description='Inertia Hub': trailerAxle1.JHub_kgm2 [-]"; p212 "Inertia Side Shaft [kgm^2] export=true name=JSideShft_kgm2 prio=1 dataSetName=axle_dummy dataClassType=axle dataClassName=$dataClassNameAxle$ moduleXmlReference=$moduleXmlReferenceAxle$ unit='kgm^2' description='Inertia Side Shaft': trailerAxle1.JSideShft_kgm2 [kgm²]"; p213 "Ratio Differential Gear [-] export=true name=iDiff prio=1 dataSetName=axle_dummy dataClassType=axle dataClassName=$dataClassNameAxle$ moduleXmlReference=$moduleXmlReferenceAxle$ unit='-' description='Ratio Differential Gear': trailerAxle2.iDiff [-]"; p214 "Is driven Axle? [-] export=true name=isDriven prio=1 dataSetName=axle_dummy dataClassType=axle dataClassName=$dataClassNameAxle$ moduleXmlReference=$moduleXmlReferenceAxle$ unit='-' description='Is Driven Axle': trailerAxle2.isDriven [-]"; p215 "Is rear Axle? [-] export=true name=isRearAxle prio=1 dataSetName=axle_dummy dataClassType=axle dataClassName=$dataClassNameAxle$ moduleXmlReference=$moduleXmlReferenceAxle$ unit='-' description='Is Rear Axle': trailerAxle2.isRearAxle [-]"; p216 "Inertia Brake Disc  [kgm^2] export=true name=JBrakeDisc_kgm2 prio=1 dataSetName=brk_dummy dataClassType=brk dataClassName=$dataClassNameBrk$ moduleXmlReference=$moduleXmlReferenceBrk$ unit='kgm^2' description='Inertia Brake Disc': trailerAxle2.JBrakeDisc_kgm2 [kgm²]"; p217 "Inertia Hub  [kgm^2] export=true name=JHub_kgm2 prio=1 dataSetName=brk_dummy dataClassType=brk dataClassName=$dataClassNameBrk$ moduleXmlReference=$moduleXmlReferenceBrk$ unit='kgm^2' description='Inertia Hub': trailerAxle2.JHub_kgm2 [-]"; p218 "Inertia Side Shaft [kgm^2] export=true name=JSideShft_kgm2 prio=1 dataSetName=axle_dummy dataClassType=axle dataClassName=$dataClassNameAxle$ moduleXmlReference=$moduleXmlReferenceAxle$ unit='kgm^2' description='Inertia Side Shaft': trailerAxle2.JSideShft_kgm2 [kgm²]"; p219 "Ratio Differential Gear [-] export=true name=iDiff prio=1 dataSetName=axle_dummy dataClassType=axle dataClassName=$dataClassNameAxle$ moduleXmlReference=$moduleXmlReferenceAxle$ unit='-' description='Ratio Differential Gear': trailerAxle3.iDiff [-]"; p220 "Is driven Axle? [-] export=true name=isDriven prio=1 dataSetName=axle_dummy dataClassType=axle dataClassName=$dataClassNameAxle$ moduleXmlReference=$moduleXmlReferenceAxle$ unit='-' description='Is Driven Axle': trailerAxle3.isDriven [-]"; p221 "Is rear Axle? [-] export=true name=isRearAxle prio=1 dataSetName=axle_dummy dataClassType=axle dataClassName=$dataClassNameAxle$ moduleXmlReference=$moduleXmlReferenceAxle$ unit='-' description='Is Rear Axle': trailerAxle3.isRearAxle [-]"; p222 "Inertia Brake Disc  [kgm^2] export=true name=JBrakeDisc_kgm2 prio=1 dataSetName=brk_dummy dataClassType=brk dataClassName=$dataClassNameBrk$ moduleXmlReference=$moduleXmlReferenceBrk$ unit='kgm^2' description='Inertia Brake Disc': trailerAxle3.JBrakeDisc_kgm2 [kgm²]"; p223 "Inertia Hub  [kgm^2] export=true name=JHub_kgm2 prio=1 dataSetName=brk_dummy dataClassType=brk dataClassName=$dataClassNameBrk$ moduleXmlReference=$moduleXmlReferenceBrk$ unit='kgm^2' description='Inertia Hub': trailerAxle3.JHub_kgm2 [-]"; p224 "Inertia Side Shaft [kgm^2] export=true name=JSideShft_kgm2 prio=1 dataSetName=axle_dummy dataClassType=axle dataClassName=$dataClassNameAxle$ moduleXmlReference=$moduleXmlReferenceAxle$ unit='kgm^2' description='Inertia Side Shaft': trailerAxle3.JSideShft_kgm2 [kgm²]"; p225 "Inertia Complete Transfer Case export=true name=JTfc_kgm2 prio=1 dataSetName=tfc_dummy dataClassType=tfc dataClassName=tfc unit='kgm^2' description='Inertia Complete Transfer Case': transferCaseA1.JTfc_kgm2 [kgm²]"; p226 "State Transfer Case export=true name=stTrfGrBoxHi prio=1 dataSetName=tfc_dummy dataClassType=tfc dataClassName=tfc unit='-' description='State Transfer Case': transferCaseA1.stTrfGrBoxHi [-]"; p227 "Air Drag Coefficient multiplied with Reference Area [m^2] export=true name=aeroCdA_m2 prio=1 dataSetName=aero_dummy dataClassType=aero dataClassName=aero unit='m^2' description='Air Drag Coefficient multiplied with Reference Area': vehicle.aeroCdA_m2 [-]"; p228 "Air Density [kg/m^3] export=true name=aeroRhoAirDensity_kgpm3 prio=1 dataSetName=aero_dummy dataClassType=aero dataClassName=aero unit='kg/m^3' description='Air Density ': vehicle.aeroRhoAirDensity_kgpm3 [-]"; p229 "number_of_weights export=true name=number_of_weights prio=1 dataSetName=massLoad_dummy dataClassType=massLoad dataClassName=massLoad unit=- description='number_of_weights': vehicle.number_of_weights [-]"; p230 "startGCW_kg export=true name=startGCW_kg prio=1 dataSetName=mass_dummy dataClassType=mass dataClassName=mass unit=kg description='startGCW_kg': vehicle.startGCW_kg [kg]"; p231 "Percentage Rolling Resistance (Rolling Resistance Coefficient) [%] export=true name=fRollCoeff prio=1 dataSetName=wheel_dummy dataClassType=wheel dataClassName=$dataClassNameWheel$ moduleXmlReference=$moduleXmlReferenceWheel$ unit='%' description='Percentage Rolling Resistance (Rolling Resistance Coefficient)': wheel_a1.fRollCoeff [-]"; p232 "Inertia Single Wheel [kgm^2] export=true name=JWheel_kgm2 prio=1 dataSetName=wheel_dummy dataClassType=wheel dataClassName=$dataClassNameWheel$ moduleXmlReference=$moduleXmlReferenceWheel$ unit='kgm^2' description='Inertia Single Wheel': wheel_a1.JWheel_kgm2 [kgm²]"; p233 "Dynamic Wheel Radius [m] export=true name=rDyn_m prio=1 dataSetName=wheel_dummy dataClassType=wheel dataClassName=$dataClassNameWheel$ moduleXmlReference=$moduleXmlReferenceWheel$ unit='m' description='Dynamic Wheel Radius': wheel_a1.rDyn_m [-]"; p234 "Percentage Rolling Resistance (Rolling Resistance Coefficient) [%] export=true name=fRollCoeff prio=1 dataSetName=wheel_dummy dataClassType=wheel dataClassName=$dataClassNameWheel$ moduleXmlReference=$moduleXmlReferenceWheel$ unit='%' description='Percentage Rolling Resistance (Rolling Resistance Coefficient)': wheel_a2.fRollCoeff [-]"; p235 "Inertia Single Wheel [kgm^2] export=true name=JWheel_kgm2 prio=1 dataSetName=wheel_dummy dataClassType=wheel dataClassName=$dataClassNameWheel$ moduleXmlReference=$moduleXmlReferenceWheel$ unit='kgm^2' description='Inertia Single Wheel': wheel_a2.JWheel_kgm2 [kgm²]"; p236 "Dynamic Wheel Radius [m] export=true name=rDyn_m prio=1 dataSetName=wheel_dummy dataClassType=wheel dataClassName=$dataClassNameWheel$ moduleXmlReference=$moduleXmlReferenceWheel$ unit='m' description='Dynamic Wheel Radius': wheel_a2.rDyn_m [-]"; p237 "Percentage Rolling Resistance (Rolling Resistance Coefficient) [%] export=true name=fRollCoeff prio=1 dataSetName=wheel_dummy dataClassType=wheel dataClassName=$dataClassNameWheel$ moduleXmlReference=$moduleXmlReferenceWheel$ unit='%' description='Percentage Rolling Resistance (Rolling Resistance Coefficient)': wheel_a3.fRollCoeff [-]"; p238 "Inertia Single Wheel [kgm^2] export=true name=JWheel_kgm2 prio=1 dataSetName=wheel_dummy dataClassType=wheel dataClassName=$dataClassNameWheel$ moduleXmlReference=$moduleXmlReferenceWheel$ unit='kgm^2' description='Inertia Single Wheel': wheel_a3.JWheel_kgm2 [kgm²]"; p239 "Dynamic Wheel Radius [m] export=true name=rDyn_m prio=1 dataSetName=wheel_dummy dataClassType=wheel dataClassName=$dataClassNameWheel$ moduleXmlReference=$moduleXmlReferenceWheel$ unit='m' description='Dynamic Wheel Radius': wheel_a3.rDyn_m [-]"; p240 "Percentage Rolling Resistance (Rolling Resistance Coefficient) [%] export=true name=fRollCoeff prio=1 dataSetName=wheel_dummy dataClassType=wheel dataClassName=$dataClassNameWheel$ moduleXmlReference=$moduleXmlReferenceWheel$ unit='%' description='Percentage Rolling Resistance (Rolling Resistance Coefficient)': wheel_a4.fRollCoeff [-]"; p241 "Inertia Single Wheel [kgm^2] export=true name=JWheel_kgm2 prio=1 dataSetName=wheel_dummy dataClassType=wheel dataClassName=$dataClassNameWheel$ moduleXmlReference=$moduleXmlReferenceWheel$ unit='kgm^2' description='Inertia Single Wheel': wheel_a4.JWheel_kgm2 [kgm²]"; p242 "Dynamic Wheel Radius [m] export=true name=rDyn_m prio=1 dataSetName=wheel_dummy dataClassType=wheel dataClassName=$dataClassNameWheel$ moduleXmlReference=$moduleXmlReferenceWheel$ unit='m' description='Dynamic Wheel Radius': wheel_a4.rDyn_m [-]"; p243 "Percentage Rolling Resistance (Rolling Resistance Coefficient) [%] export=true name=fRollCoeff prio=1 dataSetName=wheel_dummy dataClassType=wheel dataClassName=$dataClassNameWheel$ moduleXmlReference=$moduleXmlReferenceWheel$ unit='%' description='Percentage Rolling Resistance (Rolling Resistance Coefficient)': wheelTrailer_a1.fRollCoeff [-]"; p244 "Inertia Single Wheel [kgm^2] export=true name=JWheel_kgm2 prio=1 dataSetName=wheel_dummy dataClassType=wheel dataClassName=$dataClassNameWheel$ moduleXmlReference=$moduleXmlReferenceWheel$ unit='kgm^2' description='Inertia Single Wheel': wheelTrailer_a1.JWheel_kgm2 [kgm²]"; p245 "Dynamic Wheel Radius [m] export=true name=rDyn_m prio=1 dataSetName=wheel_dummy dataClassType=wheel dataClassName=$dataClassNameWheel$ moduleXmlReference=$moduleXmlReferenceWheel$ unit='m' description='Dynamic Wheel Radius': wheelTrailer_a1.rDyn_m [-]"; p246 "Percentage Rolling Resistance (Rolling Resistance Coefficient) [%] export=true name=fRollCoeff prio=1 dataSetName=wheel_dummy dataClassType=wheel dataClassName=$dataClassNameWheel$ moduleXmlReference=$moduleXmlReferenceWheel$ unit='%' description='Percentage Rolling Resistance (Rolling Resistance Coefficient)': wheelTrailer_a2.fRollCoeff [-]"; p247 "Inertia Single Wheel [kgm^2] export=true name=JWheel_kgm2 prio=1 dataSetName=wheel_dummy dataClassType=wheel dataClassName=$dataClassNameWheel$ moduleXmlReference=$moduleXmlReferenceWheel$ unit='kgm^2' description='Inertia Single Wheel': wheelTrailer_a2.JWheel_kgm2 [kgm²]"; p248 "Dynamic Wheel Radius [m] export=true name=rDyn_m prio=1 dataSetName=wheel_dummy dataClassType=wheel dataClassName=$dataClassNameWheel$ moduleXmlReference=$moduleXmlReferenceWheel$ unit='m' description='Dynamic Wheel Radius': wheelTrailer_a2.rDyn_m [-]"; p249 "Percentage Rolling Resistance (Rolling Resistance Coefficient) [%] export=true name=fRollCoeff prio=1 dataSetName=wheel_dummy dataClassType=wheel dataClassName=$dataClassNameWheel$ moduleXmlReference=$moduleXmlReferenceWheel$ unit='%' description='Percentage Rolling Resistance (Rolling Resistance Coefficient)': wheelTrailer_a3.fRollCoeff [-]"; p250 "Inertia Single Wheel [kgm^2] export=true name=JWheel_kgm2 prio=1 dataSetName=wheel_dummy dataClassType=wheel dataClassName=$dataClassNameWheel$ moduleXmlReference=$moduleXmlReferenceWheel$ unit='kgm^2' description='Inertia Single Wheel': wheelTrailer_a3.JWheel_kgm2 [kgm²]"; p251 "Dynamic Wheel Radius [m] export=true name=rDyn_m prio=1 dataSetName=wheel_dummy dataClassType=wheel dataClassName=$dataClassNameWheel$ moduleXmlReference=$moduleXmlReferenceWheel$ unit='m' description='Dynamic Wheel Radius': wheelTrailer_a3.rDyn_m [-]"; p252 "Dimension Generic Wheel Loss Torque Map export=true name=genericWheelLoss_dim prio=81 dataSetName=mecConsumers_dummy dataClassType=mecConsumers dataClassName=mecConsumers unit='' description='Dimension Generic Wheel Loss Torque Map': driveTorqueBypass1.genericWheelLoss.genericWheelLoss_dim [-]"; p253 "Dimension Generic Vehicle Loss Force Map export=true name=genericVehicleLoss_dim prio=91 dataSetName=mecConsumers_dummy dataClassType=mecConsumers dataClassName=mecConsumers unit='' description='Dimension Generic Vehicle Loss Force Map': vehicle.genericVehicleLoss.genericVehicleLoss_dim [-]"; p254 "Dimension Axle Loss Torque Map [-] export=true name=axleLoss_dim prio=1 dataSetName=axle_dummy dataClassType=axle dataClassName=$dataClassNameAxle$ moduleXmlReference=$moduleXmlReferenceAxle$ unit='-' description='Dimension Axle Loss Torque Map': axle1.axleLoss_dim [-]"; p255 "Rear Axle Loss Map [Nm] export=true name=axleLoss_map_torqueAxleIn_Nm prio=1 dataSetName=axle_dummy dataClassType=axle dataClassName=$dataClassNameAxle$ moduleXmlReference=$moduleXmlReferenceAxle$ unit='Nm' description='Rear Axle Loss Map ': axle1.axleLoss_map_torqueAxleIn_Nm [-]"; p256 "Axle Speed for Loss Torque Map [rpm] export=true name=axleLoss_x_speedAxleOut_rpm prio=1 dataSetName=axle_dummy dataClassType=axle dataClassName=$dataClassNameAxle$ moduleXmlReference=$moduleXmlReferenceAxle$ unit='rpm' description='Axle Speed for Loss Torque Map': axle1.axleLoss_x_speedAxleOut_rpm [-]"; p257 "Input Axle Torque for Loss Torque Map [Nm] export=true name=axleLoss_y_torqueAxleIn_Nm prio=1 dataSetName=axle_dummy dataClassType=axle dataClassName=$dataClassNameAxle$ moduleXmlReference=$moduleXmlReferenceAxle$ unit='Nm' description='Input Axle Torque for Loss Torque Map': axle1.axleLoss_y_torqueAxleIn_Nm [-]"; p258 "Dimension Axle Loss Torque Map [-] export=true name=axleLoss_dim prio=1 dataSetName=axle_dummy dataClassType=axle dataClassName=$dataClassNameAxle$ moduleXmlReference=$moduleXmlReferenceAxle$ unit='-' description='Dimension Axle Loss Torque Map': axle2.axleLoss_dim [-]"; p259 "Rear Axle Loss Map [Nm] export=true name=axleLoss_map_torqueAxleIn_Nm prio=1 dataSetName=axle_dummy dataClassType=axle dataClassName=$dataClassNameAxle$ moduleXmlReference=$moduleXmlReferenceAxle$ unit='Nm' description='Rear Axle Loss Map ': axle2.axleLoss_map_torqueAxleIn_Nm [-]"; p260 "Axle Speed for Loss Torque Map [rpm] export=true name=axleLoss_x_speedAxleOut_rpm prio=1 dataSetName=axle_dummy dataClassType=axle dataClassName=$dataClassNameAxle$ moduleXmlReference=$moduleXmlReferenceAxle$ unit='rpm' description='Axle Speed for Loss Torque Map': axle2.axleLoss_x_speedAxleOut_rpm [-]"; p261 "Input Axle Torque for Loss Torque Map [Nm] export=true name=axleLoss_y_torqueAxleIn_Nm prio=1 dataSetName=axle_dummy dataClassType=axle dataClassName=$dataClassNameAxle$ moduleXmlReference=$moduleXmlReferenceAxle$ unit='Nm' description='Input Axle Torque for Loss Torque Map': axle2.axleLoss_y_torqueAxleIn_Nm [-]"; p262 "Dimension Axle Loss Torque Map [-] export=true name=axleLoss_dim prio=1 dataSetName=axle_dummy dataClassType=axle dataClassName=$dataClassNameAxle$ moduleXmlReference=$moduleXmlReferenceAxle$ unit='-' description='Dimension Axle Loss Torque Map': axle3.axleLoss_dim [-]"; p263 "Rear Axle Loss Map [Nm] export=true name=axleLoss_map_torqueAxleIn_Nm prio=1 dataSetName=axle_dummy dataClassType=axle dataClassName=$dataClassNameAxle$ moduleXmlReference=$moduleXmlReferenceAxle$ unit='Nm' description='Rear Axle Loss Map ': axle3.axleLoss_map_torqueAxleIn_Nm [-]"; p264 "Axle Speed for Loss Torque Map [rpm] export=true name=axleLoss_x_speedAxleOut_rpm prio=1 dataSetName=axle_dummy dataClassType=axle dataClassName=$dataClassNameAxle$ moduleXmlReference=$moduleXmlReferenceAxle$ unit='rpm' description='Axle Speed for Loss Torque Map': axle3.axleLoss_x_speedAxleOut_rpm [-]"; p265 "Input Axle Torque for Loss Torque Map [Nm] export=true name=axleLoss_y_torqueAxleIn_Nm prio=1 dataSetName=axle_dummy dataClassType=axle dataClassName=$dataClassNameAxle$ moduleXmlReference=$moduleXmlReferenceAxle$ unit='Nm' description='Input Axle Torque for Loss Torque Map': axle3.axleLoss_y_torqueAxleIn_Nm [-]"; p266 "Dimension Axle Loss Torque Map [-] export=true name=axleLoss_dim prio=1 dataSetName=axle_dummy dataClassType=axle dataClassName=$dataClassNameAxle$ moduleXmlReference=$moduleXmlReferenceAxle$ unit='-' description='Dimension Axle Loss Torque Map': axle4.axleLoss_dim [-]"; p267 "Rear Axle Loss Map [Nm] export=true name=axleLoss_map_torqueAxleIn_Nm prio=1 dataSetName=axle_dummy dataClassType=axle dataClassName=$dataClassNameAxle$ moduleXmlReference=$moduleXmlReferenceAxle$ unit='Nm' description='Rear Axle Loss Map ': axle4.axleLoss_map_torqueAxleIn_Nm [-]"; p268 "Axle Speed for Loss Torque Map [rpm] export=true name=axleLoss_x_speedAxleOut_rpm prio=1 dataSetName=axle_dummy dataClassType=axle dataClassName=$dataClassNameAxle$ moduleXmlReference=$moduleXmlReferenceAxle$ unit='rpm' description='Axle Speed for Loss Torque Map': axle4.axleLoss_x_speedAxleOut_rpm [-]"; p269 "Input Axle Torque for Loss Torque Map [Nm] export=true name=axleLoss_y_torqueAxleIn_Nm prio=1 dataSetName=axle_dummy dataClassType=axle dataClassName=$dataClassNameAxle$ moduleXmlReference=$moduleXmlReferenceAxle$ unit='Nm' description='Input Axle Torque for Loss Torque Map': axle4.axleLoss_y_torqueAxleIn_Nm [-]"; p270 "Dimension propeller shaft Loss Torque Map  [-] export=true name=shtLoss_dim prio=1 dataSetName=sht_dummy dataClassType=sht dataClassName=$dataClassNamePropShaft$ unit='-' description='Dimension propeller shaft Loss Torque Map': propShaft_front.shtLoss_dim [-]"; p271 "Loss Torque Map Propeller Shaft [Nm] export=true name=shtLoss_map_torqueShtIn_Nm prio=1 dataSetName=sht_dummy dataClassType=sht dataClassName=$dataClassNamePropShaft$ unit='kgm^2' description='Loss Torque Map Propeller Shaft': propShaft_front.shtLoss_map_torqueShtIn_Nm [-]"; p272 "Speed Propeller Shaft for Loss Torque Map [rpm] export=true name=shtLoss_x_speedShtIn_rpm prio=1 dataSetName=sht_dummy dataClassType=sht dataClassName=$dataClassNamePropShaft$ unit='kgm^2' description='Speed Propeller Shaft for Loss Torque Map': propShaft_front.shtLoss_x_speedShtIn_rpm [-]"; p273 "Input Torque Propeller Shaft for Loss Torque Map [Nm] export=true name=shtLoss_y_torqueShtIn_Nm prio=1 dataSetName=sht_dummy dataClassType=sht dataClassName=$dataClassNamePropShaft$ unit='kgm^2' description='Input Torque Propeller Shaft for Loss Torque Map': propShaft_front.shtLoss_y_torqueShtIn_Nm [-]"; p274 "Dimension propeller shaft Loss Torque Map  [-] export=true name=shtLoss_dim prio=1 dataSetName=sht_dummy dataClassType=sht dataClassName=$dataClassNamePropShaft$ unit='-' description='Dimension propeller shaft Loss Torque Map': propShaft_rear.shtLoss_dim [-]"; p275 "Loss Torque Map Propeller Shaft [Nm] export=true name=shtLoss_map_torqueShtIn_Nm prio=1 dataSetName=sht_dummy dataClassType=sht dataClassName=$dataClassNamePropShaft$ unit='kgm^2' description='Loss Torque Map Propeller Shaft': propShaft_rear.shtLoss_map_torqueShtIn_Nm [-]"; p276 "Speed Propeller Shaft for Loss Torque Map [rpm] export=true name=shtLoss_x_speedShtIn_rpm prio=1 dataSetName=sht_dummy dataClassType=sht dataClassName=$dataClassNamePropShaft$ unit='kgm^2' description='Speed Propeller Shaft for Loss Torque Map': propShaft_rear.shtLoss_x_speedShtIn_rpm [-]"; p277 "Input Torque Propeller Shaft for Loss Torque Map [Nm] export=true name=shtLoss_y_torqueShtIn_Nm prio=1 dataSetName=sht_dummy dataClassType=sht dataClassName=$dataClassNamePropShaft$ unit='kgm^2' description='Input Torque Propeller Shaft for Loss Torque Map': propShaft_rear.shtLoss_y_torqueShtIn_Nm [-]"; p278 "Dimension Axle Loss Torque Map [-] export=true name=axleLoss_dim prio=1 dataSetName=axle_dummy dataClassType=axle dataClassName=$dataClassNameAxle$ moduleXmlReference=$moduleXmlReferenceAxle$ unit='-' description='Dimension Axle Loss Torque Map': trailerAxle1.axleLoss_dim [-]"; p279 "Rear Axle Loss Map [Nm] export=true name=axleLoss_map_torqueAxleIn_Nm prio=1 dataSetName=axle_dummy dataClassType=axle dataClassName=$dataClassNameAxle$ moduleXmlReference=$moduleXmlReferenceAxle$ unit='Nm' description='Rear Axle Loss Map ': trailerAxle1.axleLoss_map_torqueAxleIn_Nm [-]"; p280 "Axle Speed for Loss Torque Map [rpm] export=true name=axleLoss_x_speedAxleOut_rpm prio=1 dataSetName=axle_dummy dataClassType=axle dataClassName=$dataClassNameAxle$ moduleXmlReference=$moduleXmlReferenceAxle$ unit='rpm' description='Axle Speed for Loss Torque Map': trailerAxle1.axleLoss_x_speedAxleOut_rpm [-]"; p281 "Input Axle Torque for Loss Torque Map [Nm] export=true name=axleLoss_y_torqueAxleIn_Nm prio=1 dataSetName=axle_dummy dataClassType=axle dataClassName=$dataClassNameAxle$ moduleXmlReference=$moduleXmlReferenceAxle$ unit='Nm' description='Input Axle Torque for Loss Torque Map': trailerAxle1.axleLoss_y_torqueAxleIn_Nm [-]"; p282 "Dimension Axle Loss Torque Map [-] export=true name=axleLoss_dim prio=1 dataSetName=axle_dummy dataClassType=axle dataClassName=$dataClassNameAxle$ moduleXmlReference=$moduleXmlReferenceAxle$ unit='-' description='Dimension Axle Loss Torque Map': trailerAxle2.axleLoss_dim [-]"; p283 "Rear Axle Loss Map [Nm] export=true name=axleLoss_map_torqueAxleIn_Nm prio=1 dataSetName=axle_dummy dataClassType=axle dataClassName=$dataClassNameAxle$ moduleXmlReference=$moduleXmlReferenceAxle$ unit='Nm' description='Rear Axle Loss Map ': trailerAxle2.axleLoss_map_torqueAxleIn_Nm [-]"; p284 "Axle Speed for Loss Torque Map [rpm] export=true name=axleLoss_x_speedAxleOut_rpm prio=1 dataSetName=axle_dummy dataClassType=axle dataClassName=$dataClassNameAxle$ moduleXmlReference=$moduleXmlReferenceAxle$ unit='rpm' description='Axle Speed for Loss Torque Map': trailerAxle2.axleLoss_x_speedAxleOut_rpm [-]"; p285 "Input Axle Torque for Loss Torque Map [Nm] export=true name=axleLoss_y_torqueAxleIn_Nm prio=1 dataSetName=axle_dummy dataClassType=axle dataClassName=$dataClassNameAxle$ moduleXmlReference=$moduleXmlReferenceAxle$ unit='Nm' description='Input Axle Torque for Loss Torque Map': trailerAxle2.axleLoss_y_torqueAxleIn_Nm [-]"; p286 "Dimension Axle Loss Torque Map [-] export=true name=axleLoss_dim prio=1 dataSetName=axle_dummy dataClassType=axle dataClassName=$dataClassNameAxle$ moduleXmlReference=$moduleXmlReferenceAxle$ unit='-' description='Dimension Axle Loss Torque Map': trailerAxle3.axleLoss_dim [-]"; p287 "Rear Axle Loss Map [Nm] export=true name=axleLoss_map_torqueAxleIn_Nm prio=1 dataSetName=axle_dummy dataClassType=axle dataClassName=$dataClassNameAxle$ moduleXmlReference=$moduleXmlReferenceAxle$ unit='Nm' description='Rear Axle Loss Map ': trailerAxle3.axleLoss_map_torqueAxleIn_Nm [-]"; p288 "Axle Speed for Loss Torque Map [rpm] export=true name=axleLoss_x_speedAxleOut_rpm prio=1 dataSetName=axle_dummy dataClassType=axle dataClassName=$dataClassNameAxle$ moduleXmlReference=$moduleXmlReferenceAxle$ unit='rpm' description='Axle Speed for Loss Torque Map': trailerAxle3.axleLoss_x_speedAxleOut_rpm [-]"; p289 "Input Axle Torque for Loss Torque Map [Nm] export=true name=axleLoss_y_torqueAxleIn_Nm prio=1 dataSetName=axle_dummy dataClassType=axle dataClassName=$dataClassNameAxle$ moduleXmlReference=$moduleXmlReferenceAxle$ unit='Nm' description='Input Axle Torque for Loss Torque Map': trailerAxle3.axleLoss_y_torqueAxleIn_Nm [-]"; p290 "Gear Ratio Transfer Case export=true name=iTfc prio=1 dataSetName=tfc_dummy dataClassType=tfc dataClassName=tfc unit='-' description='Gear Ratio Transfer Case': transferCaseA1.iTfc [-]"; p291 "Dimension Loss Torque Map Transfer Case export=true name=tfcLoss_dim prio=1 dataSetName=tfc_dummy dataClassType=tfc dataClassName=tfc unit='-' description='Dimension Loss Torque Map Transfer Case': transferCaseA1.tfcLoss_dim [-]"; p292 "Loss Torque Map Transfer Case export=true name=tfcLoss_map_torqueTfcIn_Nm prio=1 dataSetName=tfc_dummy dataClassType=tfc dataClassName=tfc unit='Nm' description='Loss Torque Map Transfer Case': transferCaseA1.tfcLoss_map_torqueTfcIn_Nm [Nm]"; p293 "Input Speed for Loss Torque Map Transfer Case export=true name=tfcLoss_x_speedTfcIn_rpm prio=1 dataSetName=tfc_dummy dataClassType=tfc dataClassName=tfc unit='rpm' description='Output Speed for Loss Torque Map Transfer Case': transferCaseA1.tfcLoss_x_speedTfcIn_rpm [-]"; p294 "Input Torque for Loss Torque Map Transfer Case export=true name=tfcLoss_y_torqueTfcIn_Nm prio=1 dataSetName=tfc_dummy dataClassType=tfc dataClassName=tfc unit='Nm' description='Input Torque for Loss Torque Map Transfer Case': transferCaseA1.tfcLoss_y_torqueTfcIn_Nm [-]"; p295 "Torque Distribution Transfer Case export=true name=torqueDistribution prio=1 dataSetName=tfc_dummy dataClassType=tfc dataClassName=tfc unit='-' description='Torque Distribution Transfer Case': transferCaseA1.torqueDistribution [-]"; p296 "mass_distribution export=true name=mass_distribution prio=1 dataSetName=massLoad_dummy dataClassType=massLoad dataClassName=massLoad unit=- description='Mass Distribution': vehicle.mass_distribution [-]"; p297 "Air Compressor Speed for Loss Torque Map [rpm] export=true name=genericWheelLoss_x_speed_rpm prio=82 dataSetName=mecConsumers_dummy dataClassType=mecConsumers dataClassName=mecConsumers unit='rpm' description='Generic Wheel Speed for Loss Torque Map [rpm]': driveTorqueBypass1.genericWheelLoss.genericWheelLoss_x_speed_rpm [-]"; p298 "Generic Wheel Loss Torque Map [Nm] export=true name=genericWheelLoss_map_lossTorque_Nm prio=83 dataSetName=mecConsumers_dummy dataClassType=mecConsumers dataClassName=mecConsumers unit='Nm' description='Generic Wheel Loss Torque Map [Nm]': driveTorqueBypass1.genericWheelLoss.genericWheelLoss_map_lossTorque_Nm [Nm]"; p299 "Generic Vehicle Speed for Loss Force Map [rpm] export=true name=genericVehicleLoss_x_velocity_kmh prio=92 dataSetName=mecConsumers_dummy dataClassType=mecConsumers dataClassName=mecConsumers unit='rpm' description='Generic Vehicle Speed for Loss Force Map [rpm]': vehicle.genericVehicleLoss.genericVehicleLoss_x_velocity_kmh [-]"; p300 "Generic Vehicle Loss Force Map [Nm] export=true name=genericVehicleLoss_map_loss_N prio=93 dataSetName=mecConsumers_dummy dataClassType=mecConsumers dataClassName=mecConsumers unit='Nm' description='Generic Vehicle Loss Force Map [Nm]': vehicle.genericVehicleLoss.genericVehicleLoss_map_loss_N [Nm]"
  mec_tx_n2 : Outport
  mec_tx_n1 : Outport  Port=2
  mec_tx_TOut_info : Outport  Port=3
  mec_brk_Axle1_angAcc : Outport  Port=4
  mec_brk_Axle1_angPos : Outport  Port=5
  mec_brk_Axle1_angVel : Outport  Port=6
  mec_brk_Axle2_angAcc : Outport  Port=7
  mec_brk_Axle2_angPos : Outport  Port=8
  mec_brk_Axle2_angVel : Outport  Port=9
  mec_brk_Axle3_angAcc : Outport  Port=10
  mec_brk_Axle3_angPos : Outport  Port=11
  mec_brk_Axle3_angVel : Outport  Port=12
  mec_brk_Axle4_angAcc : Outport  Port=13
  mec_brk_Axle4_angPos : Outport  Port=14
  mec_brk_Axle4_angVel : Outport  Port=15
  mec_brk_TrailerAxle1_angAcc : Outport  Port=16
  mec_brk_TrailerAxle1_angPos : Outport  Port=17
  mec_brk_TrailerAxle1_angVel : Outport  Port=18
  mec_brk_TrailerAxle2_angAcc : Outport  Port=19
  mec_brk_TrailerAxle2_angPos : Outport  Port=20
  mec_brk_TrailerAxle2_angVel : Outport  Port=21
  mec_brk_TrailerAxle3_angAcc : Outport  Port=22
  mec_brk_TrailerAxle3_angPos : Outport  Port=23
  mec_brk_TrailerAxle3_angVel : Outport  Port=24
  mec_brk_Axle1_omBrk_info : Outport  Port=25
  mec_brk_Axle1_omIn_info : Outport  Port=26
  mec_brk_Axle1_TiBrk_info : Outport  Port=27
  mec_brk_Axle1_TiLoss_info : Outport  Port=28
  mec_brk_Axle1_TIn_info : Outport  Port=29
  mec_brk_Axle2_omIn_info : Outport  Port=30
  mec_brk_Axle2_TiBrk_info : Outport  Port=31
  mec_brk_Axle2_TiLoss_info : Outport  Port=32
  mec_brk_Axle2_TIn_info : Outport  Port=33
  mec_brk_Axle3_omIn_info : Outport  Port=34
  mec_brk_Axle3_TiBrk_info : Outport  Port=35
  mec_brk_Axle3_TiLoss_info : Outport  Port=36
  mec_brk_Axle3_TIn_info : Outport  Port=37
  mec_brk_Axle4_omIn_info : Outport  Port=38
  mec_brk_Axle4_TiBrk_info : Outport  Port=39
  mec_brk_Axle4_TiLoss_info : Outport  Port=40
  mec_brk_Axle4_TIn_info : Outport  Port=41
  mec_brk_TrailerAxle1_omIn_info : Outport  Port=42
  mec_brk_TrailerAxle1_TiBrk_info : Outport  Port=43
  mec_brk_TrailerAxle1_TiLoss_info : Outport  Port=44
  mec_brk_TrailerAxle1_TIn_info : Outport  Port=45
  mec_brk_TrailerAxle2_omIn_info : Outport  Port=46
  mec_brk_TrailerAxle2_TiBrk_info : Outport  Port=47
  mec_brk_TrailerAxle2_TiLoss_info : Outport  Port=48
  mec_brk_TrailerAxle2_TIn_info : Outport  Port=49
  mec_brk_TrailerAxle3_omIn_info : Outport  Port=50
  mec_brk_TrailerAxle3_TiBrk_info : Outport  Port=51
  mec_brk_TrailerAxle3_TiLoss_info : Outport  Port=52
  mec_brk_TrailerAxle3_TIn_info : Outport  Port=53
  mec_brk_TrailerWheel1_TiLossRollRes_info : Outport  Port=54
  mec_brk_TrailerWheel2_TiLossRollRes_info : Outport  Port=55
  mec_brk_TrailerWheel3_TiLossRollRes_info : Outport  Port=56
  mec_brk_Wheel1_TiLossRollRes_info : Outport  Port=57
  mec_brk_Wheel2_TiLossRollRes_info : Outport  Port=58
  mec_brk_Wheel3_TiLossRollRes_info : Outport  Port=59
  mec_brk_Wheel4_TiLossRollRes_info : Outport  Port=60
  mec_ret_T_info : Outport  Port=61
  mec_sht_omShtF_info : Outport  Port=62
  mec_sht_omShtR_info : Outport  Port=63
  mec_sht_TiLossShtF_info : Outport  Port=64
  mec_sht_TiLossShtR_info : Outport  Port=65
  mec_tfc_omOut_info : Outport  Port=66
  mec_tfc_TiLoss_info : Outport  Port=67
  mec_tfc_TOutFront_info : Outport  Port=68
  mec_tfc_TOutRear_info : Outport  Port=69
  mec_veh_domFW_info : Outport  Port=70
  mec_veh_dphiFW_info : Outport  Port=71
  mec_veh_FiAirDrag_info : Outport  Port=72
  mec_veh_FiGradeRes_info : Outport  Port=73
  mec_veh_FWheelTraction_info : Outport  Port=74
  mec_veh_sFW_info : Outport  Port=75
  mec_veh_TiFW_info : Outport  Port=76
  mec_veh_vehConfig_info : Outport  Port=77
  mec_wheel_Axle1_T_info : Outport  Port=78
  mec_wheel_Axle2_T_info : Outport  Port=79
  mec_wheel_Axle3_T_info : Outport  Port=80
  mec_wheel_Axle4_T_info : Outport  Port=81
  mec_wheel_TrailerAxle1_T_info : Outport  Port=82
  mec_wheel_TrailerAxle2_T_info : Outport  Port=83
  mec_wheel_TrailerAxle3_T_info : Outport  Port=84
  mec_brk_Axle1_left_angAcc : Outport  Port=85
  mec_brk_Axle1_left_angPos : Outport  Port=86
  mec_brk_Axle1_left_angVel : Outport  Port=87
  mec_brk_Axle1_right_angAcc : Outport  Port=88
  mec_brk_Axle1_right_angPos : Outport  Port=89
  mec_brk_Axle1_right_angVel : Outport  Port=90
  mec_brk_Axle2_left_angAcc : Outport  Port=91
  mec_brk_Axle2_left_angPos : Outport  Port=92
  mec_brk_Axle2_left_angVel : Outport  Port=93
  mec_brk_Axle2_right_angAcc : Outport  Port=94
  mec_brk_Axle2_right_angPos : Outport  Port=95
  mec_brk_Axle2_right_angVel : Outport  Port=96
  mec_brk_Axle3_left_angAcc : Outport  Port=97
  mec_brk_Axle3_left_angPos : Outport  Port=98
  mec_brk_Axle3_left_angVel : Outport  Port=99
  mec_brk_Axle3_right_angAcc : Outport  Port=100
  mec_brk_Axle3_right_angPos : Outport  Port=101
  mec_brk_Axle3_right_angVel : Outport  Port=102
  mec_brk_Axle4_left_angAcc : Outport  Port=103
  mec_brk_Axle4_left_angPos : Outport  Port=104
  mec_brk_Axle4_left_angVel : Outport  Port=105
  mec_brk_Axle4_right_angAcc : Outport  Port=106
  mec_brk_Axle4_right_angPos : Outport  Port=107
  mec_brk_Axle4_right_angVel : Outport  Port=108
  mec_brk_TrailerAxle1_left_angAcc : Outport  Port=109
  mec_brk_TrailerAxle1_left_angPos : Outport  Port=110
  mec_brk_TrailerAxle1_left_angVel : Outport  Port=111
  mec_brk_TrailerAxle1_right_angAcc : Outport  Port=112
  mec_brk_TrailerAxle1_right_angPos : Outport  Port=113
  mec_brk_TrailerAxle1_right_angVel : Outport  Port=114
  mec_brk_TrailerAxle2_left_angAcc : Outport  Port=115
  mec_brk_TrailerAxle2_left_angPos : Outport  Port=116
  mec_brk_TrailerAxle2_left_angVel : Outport  Port=117
  mec_brk_TrailerAxle2_right_angAcc : Outport  Port=118
  mec_brk_TrailerAxle2_right_angPos : Outport  Port=119
  mec_brk_TrailerAxle2_right_angVel : Outport  Port=120
  mec_brk_TrailerAxle3_left_angAcc : Outport  Port=121
  mec_brk_TrailerAxle3_left_angPos : Outport  Port=122
  mec_brk_TrailerAxle3_left_angVel : Outport  Port=123
  mec_brk_TrailerAxle3_right_angAcc : Outport  Port=124
  mec_brk_TrailerAxle3_right_angPos : Outport  Port=125
  mec_brk_TrailerAxle3_right_angVel : Outport  Port=126
  mec_ret_Retarder_angAcc : Outport  Port=127
  mec_ret_Retarder_angPos : Outport  Port=128
  mec_ret_Retarder_angVel : Outport  Port=129
  mec_veh_GenericLoss_transAcc : Outport  Port=130
  mec_veh_GenericLoss_transPos : Outport  Port=131
  mec_veh_GenericLoss_transVel : Outport  Port=132
  mec_veh_VehVelReferenceCool_velocity : Outport  Port=133
  mec_veh_VehVelReferenceUhood_velocity : Outport  Port=134
  mec_wheel_GenericLoss_angAcc : Outport  Port=135
  mec_wheel_GenericLoss_angPos : Outport  Port=136
  mec_wheel_GenericLoss_angVel : Outport  Port=137
  mec_tx_inclRoadSns : Outport  Port=138
  mec_tx_nGbOutD3Sns : Outport  Port=139
  mec_tx_nGbOutDzAwSns : Outport  Port=140
  mec_tx_nGbOutDzSfSns : Outport  Port=141
  mec_tx_nGbOutDzTuAwSns : Outport  Port=142
  mec_tx_nGbOutSns : Outport  Port=143
  mec_veh_AxleLoad1 : Outport  Port=144
  mec_veh_AxleLoad2 : Outport  Port=145
  mec_veh_AxleLoad3 : Outport  Port=146
  mec_veh_AxleLoad4 : Outport  Port=147
  mec_veh_fRollCoeffOverall : Outport  Port=148
  mec_veh_massVehicle : Outport  Port=149
  mec_veh_Payload : Outport  Port=150
  mec_veh_TotalGroCombWeight : Outport  Port=151
  mec_veh_TrailerAxleLoad1 : Outport  Port=152
  mec_veh_TrailerAxleLoad2 : Outport  Port=153
  mec_veh_TrailerAxleLoad3 : Outport  Port=154
  mec_veh_transAcc : Outport  Port=155
  mec_veh_transPos : Outport  Port=156
  mec_veh_transVel : Outport  Port=157
  mec_eng_Starter_angPos : Outport  Port=158
  mec_eng_Starter_angVel : Outport  Port=159
  mec_eng_Starter_angAcc : Outport  Port=160
  mec_eng_starter_T_info : Outport  Port=161
  mec_eng_CrankMean_angAcc : Outport  Port=162
  mec_eng_CrankMean_angPos : Outport  Port=163
  mec_eng_CrankMean_angVel : Outport  Port=164
  mec_brk_AirCompressor_angPos : Outport  Port=165
  mec_brk_AirCompressor_angVel : Outport  Port=166
  mec_brk_AirCompressor_angAcc : Outport  Port=167
  mec_eng_Consumer_angPos : Outport  Port=168
  mec_eng_Consumer_angVel : Outport  Port=169
  mec_eng_Consumer_angAcc : Outport  Port=170
  mec_eng_Generator_angPos : Outport  Port=171
  mec_eng_Generator_angVel : Outport  Port=172
  mec_eng_Generator_angAcc : Outport  Port=173
  mec_eng_MainFan_angPos : Outport  Port=174
  mec_eng_MainFan_angVel : Outport  Port=175
  mec_eng_MainFan_angAcc : Outport  Port=176
  mec_eng_MainPump_angPos : Outport  Port=177
  mec_eng_MainPump_angVel : Outport  Port=178
  mec_eng_MainPump_angAcc : Outport  Port=179
  mec_eng_EmotCrankshaft_angPos : Outport  Port=180
  mec_eng_EmotCrankshaft_angVel : Outport  Port=181
  mec_eng_EmotCrankshaft_angAcc : Outport  Port=182
  mec_eng_speedCrankshaftSegment : Outport  Port=183
  mec_eng_speedCrankshaft : Outport  Port=184
  mec_eng_speedGradCrankshaft : Outport  Port=185
  mec_eng_speedGradCrankshaftSegment : Outport  Port=186
  mec_eng_Consumer_angVel_info : Outport  Port=187
  mec_eng_Consumer_torque_info : Outport  Port=188
  mec_eng_Generator_angVel_info : Outport  Port=189
  mec_eng_Generator_torque_info : Outport  Port=190
  mec_eng_MainFan_angVel_info : Outport  Port=191
  mec_eng_MainFan_torque_info : Outport  Port=192
  mec_eng_MainPump_angVel_info : Outport  Port=193
  mec_eng_MainPump_torque_info : Outport  Port=194
  mec_brk_AirCompressor_angVel_info : Outport  Port=195
  mec_brk_AirCompressor_torque_info : Outport  Port=196
  mec_tx_TiLossIn_info : Outport  Port=197
  mec_MaxRetTrq_Cval_PT : Outport  Port=198
  mec_ActMaxRetTrqNoTemp_Cval_PT : Outport  Port=199
  mec_FuncLmpRet_Rq : Outport  Port=200
  mec_RetAct_Stat_PT : Outport  Port=201
  mec_MinRetTrqPwrUp_Stat_PT : Outport  Port=202
  mec_RetTrqCval_PT : Outport  Port=203
  mec_BrkTrqServBrk_Nm : Outport  Port=204
  wires:
  DIWA_NXT/2(Getriebeausgangsmoment_Nm) -> mec_pointmass_generic_ATvoith_std/20(mec_eng_CrankMean_torque), mec_tx_TOut_info/1  "mec_eng_CrankMean_torque"
  mec_pointmass_generic_ATvoith_std/136(mec_tx_nGbOutD3Sns) -> Memory/1, mec_tx_nGbOutD3Sns/1  "mec_tx_nGbOutD3Sns"
  Memory/1 -> DIWA_NXT/2(Getriebeausgangsdrehzahl_rpm)
  tcm_p_SK/1 -> DIWA_NXT/5(tcm_p_SK)
  tcm_p_TWB/1 -> DIWA_NXT/7(tcm_p_TWB)
  tcm_p_PB/1 -> DIWA_NXT/6(tcm_p_PB)
  tcm_p_EK/1 -> DIWA_NXT/3(tcm_p_EK)
  tcm_AKc2/1 -> DIWA_NXT/10(tcm_AKc2)
  tcm_p_TGB/1 -> DIWA_NXT/8(tcm_p_TGB)
  tcm_AKs2/1 -> DIWA_NXT/9(tcm_AKs2)
  tcm_p_DK/1 -> DIWA_NXT/4(tcm_p_DK)
  mec_pointmass_generic_ATvoith_std/126(mec_ret_Retarder_angVel) -> mec_ret_Retarder_angVel/1  "mec_ret_Retarder_angVel"
  mec_pointmass_generic_ATvoith_std/133(mec_wheel_GenericLoss_angPos) -> mec_wheel_GenericLoss_angPos/1  "mec_wheel_GenericLoss_angPos"
  mec_pointmass_generic_ATvoith_std/72(mec_veh_sFW_info) -> mec_veh_sFW_info/1  "mec_veh_sFW_info"
  mec_pointmass_generic_ATvoith_std/125(mec_ret_Retarder_angPos) -> mec_ret_Retarder_angPos/1  "mec_ret_Retarder_angPos"
  mec_pointmass_generic_ATvoith_std/128(mec_veh_GenericLoss_transPos) -> mec_veh_GenericLoss_transPos/1  "mec_veh_GenericLoss_transPos"
  mec_pointmass_generic_ATvoith_std/11(mec_brk_Axle4_angPos) -> mec_brk_Axle4_angPos/1  "mec_brk_Axle4_angPos"
  mec_pointmass_generic_ATvoith_std/124(mec_ret_Retarder_angAcc) -> mec_ret_Retarder_angAcc/1  "mec_ret_Retarder_angAcc"
  mec_pointmass_generic_ATvoith_std/134(mec_wheel_GenericLoss_angVel) -> mec_wheel_GenericLoss_angVel/1  "mec_wheel_GenericLoss_angVel"
  mec_pointmass_generic_ATvoith_std/7(mec_brk_Axle3_angAcc) -> mec_brk_Axle3_angAcc/1  "mec_brk_Axle3_angAcc"
  mec_pointmass_generic_ATvoith_std/67(mec_veh_domFW_info) -> mec_veh_domFW_info/1  "mec_veh_domFW_info"
  mec_pointmass_generic_ATvoith_std/10(mec_brk_Axle4_angAcc) -> mec_brk_Axle4_angAcc/1  "mec_brk_Axle4_angAcc"
  mec_pointmass_generic_ATvoith_std/75(mec_wheel_Axle1_T_info) -> mec_wheel_Axle1_T_info/1  "mec_wheel_Axle1_T_info"
  mec_pointmass_generic_ATvoith_std/68(mec_veh_dphiFW_info) -> mec_veh_dphiFW_info/1  "mec_veh_dphiFW_info"
  mec_pointmass_generic_ATvoith_std/69(mec_veh_FiAirDrag_info) -> mec_veh_FiAirDrag_info/1  "mec_veh_FiAirDrag_info"
  mec_pointmass_generic_ATvoith_std/76(mec_wheel_Axle2_T_info) -> mec_wheel_Axle2_T_info/1  "mec_wheel_Axle2_T_info"
  mec_pointmass_generic_ATvoith_std/12(mec_brk_Axle4_angVel) -> mec_brk_Axle4_angVel/1  "mec_brk_Axle4_angVel"
  mec_pointmass_generic_ATvoith_std/70(mec_veh_FiGradeRes_info) -> mec_veh_FiGradeRes_info/1  "mec_veh_FiGradeRes_info"
  mec_pointmass_generic_ATvoith_std/13(mec_brk_TrailerAxle1_angAcc) -> mec_brk_TrailerAxle1_angAcc/1  "mec_brk_TrailerAxle1_angAcc"
  mec_pointmass_generic_ATvoith_std/77(mec_wheel_Axle3_T_info) -> mec_wheel_Axle3_T_info/1  "mec_wheel_Axle3_T_info"
  mec_pointmass_generic_ATvoith_std/14(mec_brk_TrailerAxle1_angPos) -> mec_brk_TrailerAxle1_angPos/1  "mec_brk_TrailerAxle1_angPos"
  mec_pointmass_generic_ATvoith_std/5(mec_brk_Axle2_angPos) -> mec_brk_Axle2_angPos/1  "mec_brk_Axle2_angPos"
  mec_pointmass_generic_ATvoith_std/127(mec_veh_GenericLoss_transAcc) -> mec_veh_GenericLoss_transAcc/1  "mec_veh_GenericLoss_transAcc"
  mec_pointmass_generic_ATvoith_std/8(mec_brk_Axle3_angPos) -> mec_brk_Axle3_angPos/1  "mec_brk_Axle3_angPos"
  mec_pointmass_generic_ATvoith_std/63(mec_tfc_omOut_info) -> mec_tfc_omOut_info/1  "mec_tfc_omOut_info"
  mec_pointmass_generic_ATvoith_std/139(mec_tx_nGbOutDzTuAwSns) -> mec_tx_nGbOutDzTuAwSns/1  "mec_tx_nGbOutDzTuAwSns"
  mec_pointmass_generic_ATvoith_std/4(mec_brk_Axle2_angAcc) -> mec_brk_Axle2_angAcc/1  "mec_brk_Axle2_angAcc"
  mec_pointmass_generic_ATvoith_std/17(mec_brk_TrailerAxle2_angPos) -> mec_brk_TrailerAxle2_angPos/1  "mec_brk_TrailerAxle2_angPos"
  mec_pointmass_generic_ATvoith_std/79(mec_wheel_TrailerAxle1_T_info) -> mec_wheel_TrailerAxle1_T_info/1  "mec_wheel_TrailerAxle1_T_info"
  mec_pointmass_generic_ATvoith_std/20(mec_brk_TrailerAxle3_angPos) -> mec_brk_TrailerAxle3_angPos/1  "mec_brk_TrailerAxle3_angPos"
  mec_pointmass_generic_ATvoith_std/80(mec_wheel_TrailerAxle2_T_info) -> mec_wheel_TrailerAxle2_T_info/1  "mec_wheel_TrailerAxle2_T_info"
  mec_pointmass_generic_ATvoith_std/6(mec_brk_Axle2_angVel) -> mec_brk_Axle2_angVel/1  "mec_brk_Axle2_angVel"
  mec_pointmass_generic_ATvoith_std/81(mec_wheel_TrailerAxle3_T_info) -> mec_wheel_TrailerAxle3_T_info/1  "mec_wheel_TrailerAxle3_T_info"
  mec_pointmass_generic_ATvoith_std/15(mec_brk_TrailerAxle1_angVel) -> mec_brk_TrailerAxle1_angVel/1  "mec_brk_TrailerAxle1_angVel"
  mec_pointmass_generic_ATvoith_std/131(mec_veh_VehVelReferenceUhood_velocity) -> mec_veh_VehVelReferenceUhood_velocity/1  "mec_veh_VehVelReferenceUhood_velocity"
  mec_pointmass_generic_ATvoith_std/2(mec_brk_Axle1_angPos) -> mec_brk_Axle1_angPos/1  "mec_brk_Axle1_angPos"
  mec_pointmass_generic_ATvoith_std/132(mec_wheel_GenericLoss_angAcc) -> mec_wheel_GenericLoss_angAcc/1  "mec_wheel_GenericLoss_angAcc"
  mec_pointmass_generic_ATvoith_std/140(mec_tx_nGbOutSns) -> mec_tx_nGbOutSns/1  "mec_tx_nGbOutSns"
  mec_pointmass_generic_ATvoith_std/135(mec_tx_inclRoadSns) -> mec_tx_inclRoadSns/1  "mec_tx_inclRoadSns"
  mec_pointmass_generic_ATvoith_std/78(mec_wheel_Axle4_T_info) -> mec_wheel_Axle4_T_info/1  "mec_wheel_Axle4_T_info"
  mec_pointmass_generic_ATvoith_std/19(mec_brk_TrailerAxle3_angAcc) -> mec_brk_TrailerAxle3_angAcc/1  "mec_brk_TrailerAxle3_angAcc"
  mec_pointmass_generic_ATvoith_std/129(mec_veh_GenericLoss_transVel) -> mec_veh_GenericLoss_transVel/1  "mec_veh_GenericLoss_transVel"
  mec_pointmass_generic_ATvoith_std/18(mec_brk_TrailerAxle2_angVel) -> mec_brk_TrailerAxle2_angVel/1  "mec_brk_TrailerAxle2_angVel"
  mec_pointmass_generic_ATvoith_std/16(mec_brk_TrailerAxle2_angAcc) -> mec_brk_TrailerAxle2_angAcc/1  "mec_brk_TrailerAxle2_angAcc"
  mec_pointmass_generic_ATvoith_std/74(mec_veh_vehConfig_info) -> mec_veh_vehConfig_info/1  "mec_veh_vehConfig_info"
  mec_pointmass_generic_ATvoith_std/1(mec_brk_Axle1_angAcc) -> mec_brk_Axle1_angAcc/1  "mec_brk_Axle1_angAcc"
  mec_pointmass_generic_ATvoith_std/3(mec_brk_Axle1_angVel) -> mec_brk_Axle1_angVel/1  "mec_brk_Axle1_angVel"
  mec_pointmass_generic_ATvoith_std/21(mec_brk_TrailerAxle3_angVel) -> mec_brk_TrailerAxle3_angVel/1  "mec_brk_TrailerAxle3_angVel"
  mec_pointmass_generic_ATvoith_std/32(mec_brk_Axle3_TiBrk_info) -> mec_brk_Axle3_TiBrk_info/1  "mec_brk_Axle3_TiBrk_info"
  mec_pointmass_generic_ATvoith_std/30(mec_brk_Axle2_TIn_info) -> mec_brk_Axle2_TIn_info/1  "mec_brk_Axle2_TIn_info"
  mec_pointmass_generic_ATvoith_std/31(mec_brk_Axle3_omIn_info) -> mec_brk_Axle3_omIn_info/1  "mec_brk_Axle3_omIn_info"
  mec_pointmass_generic_ATvoith_std/33(mec_brk_Axle3_TiLoss_info) -> mec_brk_Axle3_TiLoss_info/1  "mec_brk_Axle3_TiLoss_info"
  mec_pointmass_generic_ATvoith_std/34(mec_brk_Axle3_TIn_info) -> mec_brk_Axle3_TIn_info/1  "mec_brk_Axle3_TIn_info"
  mec_pointmass_generic_ATvoith_std/36(mec_brk_Axle4_TiBrk_info) -> mec_brk_Axle4_TiBrk_info/1  "mec_brk_Axle4_TiBrk_info"
  mec_pointmass_generic_ATvoith_std/35(mec_brk_Axle4_omIn_info) -> mec_brk_Axle4_omIn_info/1  "mec_brk_Axle4_omIn_info"
  mec_pointmass_generic_ATvoith_std/38(mec_brk_Axle4_TIn_info) -> mec_brk_Axle4_TIn_info/1  "mec_brk_Axle4_TIn_info"
  mec_pointmass_generic_ATvoith_std/37(mec_brk_Axle4_TiLoss_info) -> mec_brk_Axle4_TiLoss_info/1  "mec_brk_Axle4_TiLoss_info"
  mec_pointmass_generic_ATvoith_std/39(mec_brk_TrailerAxle1_omIn_info) -> mec_brk_TrailerAxle1_omIn_info/1  "mec_brk_TrailerAxle1_omIn_info"
  mec_pointmass_generic_ATvoith_std/40(mec_brk_TrailerAxle1_TiBrk_info) -> mec_brk_TrailerAxle1_TiBrk_info/1  "mec_brk_TrailerAxle1_TiBrk_info"
  mec_pointmass_generic_ATvoith_std/41(mec_brk_TrailerAxle1_TiLoss_info) -> mec_brk_TrailerAxle1_TiLoss_info/1  "mec_brk_TrailerAxle1_TiLoss_info"
  mec_pointmass_generic_ATvoith_std/42(mec_brk_TrailerAxle1_TIn_info) -> mec_brk_TrailerAxle1_TIn_info/1  "mec_brk_TrailerAxle1_TIn_info"
  mec_pointmass_generic_ATvoith_std/44(mec_brk_TrailerAxle2_TiBrk_info) -> mec_brk_TrailerAxle2_TiBrk_info/1  "mec_brk_TrailerAxle2_TiBrk_info"
  mec_pointmass_generic_ATvoith_std/43(mec_brk_TrailerAxle2_omIn_info) -> mec_brk_TrailerAxle2_omIn_info/1  "mec_brk_TrailerAxle2_omIn_info"
  mec_pointmass_generic_ATvoith_std/46(mec_brk_TrailerAxle2_TIn_info) -> mec_brk_TrailerAxle2_TIn_info/1  "mec_brk_TrailerAxle2_TIn_info"
  mec_pointmass_generic_ATvoith_std/66(mec_tfc_TOutRear_info) -> mec_tfc_TOutRear_info/1  "mec_tfc_TOutRear_info"
  mec_pointmass_generic_ATvoith_std/62(mec_sht_TiLossShtR_info) -> mec_sht_TiLossShtR_info/1  "mec_sht_TiLossShtR_info"
  mec_pointmass_generic_ATvoith_std/49(mec_brk_TrailerAxle3_TiLoss_info) -> mec_brk_TrailerAxle3_TiLoss_info/1  "mec_brk_TrailerAxle3_TiLoss_info"
  mec_pointmass_generic_ATvoith_std/58(mec_ret_T_info) -> mec_ret_T_info/1  "mec_ret_T_info"
  mec_pointmass_generic_ATvoith_std/57(mec_brk_Wheel4_TiLossRollRes_info) -> mec_brk_Wheel4_TiLossRollRes_info/1  "mec_brk_Wheel4_TiLossRollRes_info"
  mec_pointmass_generic_ATvoith_std/55(mec_brk_Wheel2_TiLossRollRes_info) -> mec_brk_Wheel2_TiLossRollRes_info/1  "mec_brk_Wheel2_TiLossRollRes_info"
  mec_pointmass_generic_ATvoith_std/48(mec_brk_TrailerAxle3_TiBrk_info) -> mec_brk_TrailerAxle3_TiBrk_info/1  "mec_brk_TrailerAxle3_TiBrk_info"
  mec_pointmass_generic_ATvoith_std/54(mec_brk_Wheel1_TiLossRollRes_info) -> mec_brk_Wheel1_TiLossRollRes_info/1  "mec_brk_Wheel1_TiLossRollRes_info"
  mec_pointmass_generic_ATvoith_std/50(mec_brk_TrailerAxle3_TIn_info) -> mec_brk_TrailerAxle3_TIn_info/1  "mec_brk_TrailerAxle3_TIn_info"
  mec_pointmass_generic_ATvoith_std/52(mec_brk_TrailerWheel2_TiLossRollRes_info) -> mec_brk_TrailerWheel2_TiLossRollRes_info/1  "mec_brk_TrailerWheel2_TiLossRollRes_info"
  mec_pointmass_generic_ATvoith_std/56(mec_brk_Wheel3_TiLossRollRes_info) -> mec_brk_Wheel3_TiLossRollRes_info/1  "mec_brk_Wheel3_TiLossRollRes_info"
  mec_pointmass_generic_ATvoith_std/64(mec_tfc_TiLoss_info) -> mec_tfc_TiLoss_info/1  "mec_tfc_TiLoss_info"
  mec_pointmass_generic_ATvoith_std/59(mec_sht_omShtF_info) -> mec_sht_omShtF_info/1  "mec_sht_omShtF_info"
  mec_pointmass_generic_ATvoith_std/60(mec_sht_omShtR_info) -> mec_sht_omShtR_info/1  "mec_sht_omShtR_info"
  mec_pointmass_generic_ATvoith_std/45(mec_brk_TrailerAxle2_TiLoss_info) -> mec_brk_TrailerAxle2_TiLoss_info/1  "mec_brk_TrailerAxle2_TiLoss_info"
  mec_pointmass_generic_ATvoith_std/71(mec_veh_FWheelTraction_info) -> mec_veh_FWheelTraction_info/1  "mec_veh_FWheelTraction_info"
  mec_pointmass_generic_ATvoith_std/138(mec_tx_nGbOutDzSfSns) -> mec_tx_nGbOutDzSfSns/1  "mec_tx_nGbOutDzSfSns"
  mec_pointmass_generic_ATvoith_std/137(mec_tx_nGbOutDzAwSns) -> mec_tx_nGbOutDzAwSns/1  "mec_tx_nGbOutDzAwSns"
  mec_pointmass_generic_ATvoith_std/73(mec_veh_TiFW_info) -> mec_veh_TiFW_info/1  "mec_veh_TiFW_info"
  mec_pointmass_generic_ATvoith_std/9(mec_brk_Axle3_angVel) -> mec_brk_Axle3_angVel/1  "mec_brk_Axle3_angVel"
  mec_pointmass_generic_ATvoith_std/51(mec_brk_TrailerWheel1_TiLossRollRes_info) -> mec_brk_TrailerWheel1_TiLossRollRes_info/1  "mec_brk_TrailerWheel1_TiLossRollRes_info"
  mec_pointmass_generic_ATvoith_std/47(mec_brk_TrailerAxle3_omIn_info) -> mec_brk_TrailerAxle3_omIn_info/1  "mec_brk_TrailerAxle3_omIn_info"
  mec_pointmass_generic_ATvoith_std/65(mec_tfc_TOutFront_info) -> mec_tfc_TOutFront_info/1  "mec_tfc_TOutFront_info"
  mec_pointmass_generic_ATvoith_std/53(mec_brk_TrailerWheel3_TiLossRollRes_info) -> mec_brk_TrailerWheel3_TiLossRollRes_info/1  "mec_brk_TrailerWheel3_TiLossRollRes_info"
  mec_pointmass_generic_ATvoith_std/61(mec_sht_TiLossShtF_info) -> mec_sht_TiLossShtF_info/1  "mec_sht_TiLossShtF_info"
  mec_brk_Axle3_left_torque/1 -> mec_pointmass_generic_ATvoith_std/10(mec_brk_Axle3_left_torque)
  mec_brk_TrailerAxle2_left_torque/1 -> mec_pointmass_generic_ATvoith_std/16(mec_brk_TrailerAxle2_left_torque)
  mec_brk_Axle1_left_torque/1 -> mec_pointmass_generic_ATvoith_std/6(mec_brk_Axle1_left_torque)
  mec_brk_Axle2_left_torque/1 -> mec_pointmass_generic_ATvoith_std/8(mec_brk_Axle2_left_torque)
  mec_ret_Retarder_torque/1 -> mec_pointmass_generic_ATvoith_std/21(mec_ret_Retarder_torque)
  cpc_cdA_offset/1 -> mec_pointmass_generic_ATvoith_std/1(cpc_cdA_offset)
  mec_veh_GenericLoss_force/1 -> mec_pointmass_generic_ATvoith_std/22(mec_veh_GenericLoss_force)
  mec_brk_Axle4_left_torque/1 -> mec_pointmass_generic_ATvoith_std/12(mec_brk_Axle4_left_torque)
  mec_brk_TrailerAxle1_left_torque/1 -> mec_pointmass_generic_ATvoith_std/14(mec_brk_TrailerAxle1_left_torque)
  mec_wheel_GenericLoss_torque/1 -> mec_pointmass_generic_ATvoith_std/23(mec_wheel_GenericLoss_torque)
  env_road_slope_pct/1 -> mec_pointmass_generic_ATvoith_std/5(env_road_slope_pct)
  mec_pointmass_generic_ATvoith_std/28(mec_brk_Axle2_TiBrk_info) -> mec_brk_Axle2_TiBrk_info/1  "mec_brk_Axle2_TiBrk_info"
  mec_pointmass_generic_ATvoith_std/25(mec_brk_Axle1_TiLoss_info) -> mec_brk_Axle1_TiLoss_info/1  "mec_brk_Axle1_TiLoss_info"
  mec_pointmass_generic_ATvoith_std/26(mec_brk_Axle1_TIn_info) -> mec_brk_Axle1_TIn_info/1  "mec_brk_Axle1_TIn_info"
  mec_pointmass_generic_ATvoith_std/23(mec_brk_Axle1_omIn_info) -> mec_brk_Axle1_omIn_info/1  "mec_brk_Axle1_omIn_info"
  mec_pointmass_generic_ATvoith_std/22(mec_brk_Axle1_omBrk_info) -> mec_brk_Axle1_omBrk_info/1  "mec_brk_Axle1_omBrk_info"
  mec_pointmass_generic_ATvoith_std/29(mec_brk_Axle2_TiLoss_info) -> mec_brk_Axle2_TiLoss_info/1  "mec_brk_Axle2_TiLoss_info"
  mec_pointmass_generic_ATvoith_std/27(mec_brk_Axle2_omIn_info) -> mec_brk_Axle2_omIn_info/1  "mec_brk_Axle2_omIn_info"
  mec_pointmass_generic_ATvoith_std/24(mec_brk_Axle1_TiBrk_info) -> mec_brk_Axle1_TiBrk_info/1  "mec_brk_Axle1_TiBrk_info"
  Sum1/1 -> DIWA_NXT/1(Getriebeeingangsmoment_Nm)
  Product/1 -> StarterMap/1
  Constant/1 -> Product/2
  mcm_starter_on/1 -> Product1/2
  StarterMap/1 -> Sum/1
  Product3/1 -> Sum1/3
  Integrator/1 -> mec_eng_Starter_angPos/1
  Gain1/1 -> Derivative2/1, mec_eng_Starter_angVel/1, Integrator/1
  Derivative2/1 -> mec_eng_Starter_angAcc/1
  Constant1/1 -> Product3/1, Product2/1
  Product1/1 -> Product3/2, mec_eng_starter_T_info/1
  Product2/1 -> Product/1, Gain1/1
  Sum/1 -> Product1/1
  mec_eng_Starter_torque/1 -> Sum/2
  mec_pointmass_generic_ATvoith_std/130(mec_veh_VehVelReferenceCool_velocity) -> mec_veh_VehVelReferenceCool_velocity/1  "mec_veh_VehVelReferenceCool_velocity"
  DIWA_NXT/1(Motordrehzahl_rpm) -> Product2/2, Engine/8(EngineSpeed_fromDiwaGearBoxModel)
  mec_brk_AirCompressor_torque/1 -> Engine/1(mec_brk_AirCompressor_torque)
  mec_eng_Generator_torque/1 -> Engine/2(mec_eng_Generator_torque)
  mec_eng_Consumer_torque/1 -> Engine/3(mec_eng_Consumer_torque)
  mec_eng_MainFan_torque/1 -> Engine/4(mec_eng_MainFan_torque)
  mec_eng_MainPump_torque/1 -> Engine/5(mec_eng_MainPump_torque)
  Engine/26(TorqueLossEngine) -> Sum1/1
  Engine/1(mec_eng_CrankMean_angPos) -> mec_eng_CrankMean_angPos/1
  Engine/2(mec_eng_CrankMean_angVel) -> mec_eng_CrankMean_angVel/1
  Engine/3(mec_eng_CrankMean_angAcc) -> mec_eng_CrankMean_angAcc/1
  Engine/6(mec_brk_AirCompressor_angAcc) -> mec_brk_AirCompressor_angAcc/1
  Engine/5(mec_brk_AirCompressor_angVel) -> mec_brk_AirCompressor_angVel/1
  Engine/4(mec_brk_AirCompressor_angPos) -> mec_brk_AirCompressor_angPos/1
  Engine/7(mec_eng_Consumer_angPos) -> mec_eng_Consumer_angPos/1
  Engine/8(mec_eng_Consumer_angVel) -> mec_eng_Consumer_angVel/1
  Engine/9(mec_eng_Consumer_angAcc) -> mec_eng_Consumer_angAcc/1
  Engine/10(mec_eng_Generator_angPos) -> mec_eng_Generator_angPos/1
  Engine/11(mec_eng_Generator_angVel) -> mec_eng_Generator_angVel/1
  Engine/12(mec_eng_Generator_angAcc) -> mec_eng_Generator_angAcc/1
  Engine/13(mec_eng_MainFan_angPos) -> mec_eng_MainFan_angPos/1
  Engine/14(mec_eng_MainFan_angVel) -> mec_eng_MainFan_angVel/1
  Engine/15(mec_eng_MainFan_angAcc) -> mec_eng_MainFan_angAcc/1
  Engine/16(mec_eng_MainPump_angPos) -> mec_eng_MainPump_angPos/1
  Engine/17(mec_eng_MainPump_angVel) -> mec_eng_MainPump_angVel/1
  Engine/18(mec_eng_MainPump_angAcc) -> mec_eng_MainPump_angAcc/1
  Engine/22(mec_eng_speedCrankshaftSegment) -> mec_eng_speedCrankshaftSegment/1
  Engine/23(mec_eng_speedCrankshaft) -> mec_eng_speedCrankshaft/1
  Engine/24(mec_eng_speedGradCrankshaft) -> mec_eng_speedGradCrankshaft/1
  Engine/25(mec_eng_speedGradCrankshaftSegment) -> mec_eng_speedGradCrankshaftSegment/1
  mec_eng_EmotCrankshaft_torque/1 -> Engine/6(mec_eng_EmotCrankshaft_torque)
  Engine/19(mec_eng_EmotCrankshaft_angPos) -> mec_eng_EmotCrankshaft_angPos/1
  Engine/20(mec_eng_EmotCrankshaft_angVel) -> mec_eng_EmotCrankshaft_angVel/1
  Engine/21(mec_eng_EmotCrankshaft_angAcc) -> mec_eng_EmotCrankshaft_angAcc/1
  Engine/27(mec_eng_Consumer_angVel_info) -> mec_eng_Consumer_angVel_info/1
  Engine/28(mec_eng_Consumer_torque_info) -> mec_eng_Consumer_torque_info/1
  Engine/29(mec_eng_Generator_angVel_info) -> mec_eng_Generator_angVel_info/1
  Engine/30(mec_eng_Generator_torque_info) -> mec_eng_Generator_torque_info/1
  Engine/31(mec_eng_MainFan_angVel_info) -> mec_eng_MainFan_angVel_info/1
  Engine/32(mec_eng_MainFan_torque_info) -> mec_eng_MainFan_torque_info/1
  Engine/33(mec_eng_MainPump_angVel_info) -> mec_eng_MainPump_angVel_info/1
  Engine/34(mec_eng_MainPump_torque_info) -> mec_eng_MainPump_torque_info/1
  Engine/35(mec_brk_AirCompressor_angVel_info) -> mec_brk_AirCompressor_angVel_info/1
  Engine/36(mec_brk_AirCompressor_torque_info) -> mec_brk_AirCompressor_torque_info/1
  env_density/1 -> mec_pointmass_generic_ATvoith_std/3(env_density)
  env_curv_pm/1 -> mec_pointmass_generic_ATvoith_std/2(env_curv_pm)
  mec_brk_Axle1_right_torque/1 -> mec_pointmass_generic_ATvoith_std/7(mec_brk_Axle1_right_torque)
  mec_brk_Axle2_right_torque/1 -> mec_pointmass_generic_ATvoith_std/9(mec_brk_Axle2_right_torque)
  mec_brk_Axle3_right_torque/1 -> mec_pointmass_generic_ATvoith_std/11(mec_brk_Axle3_right_torque)
  mec_brk_Axle4_right_torque/1 -> mec_pointmass_generic_ATvoith_std/13(mec_brk_Axle4_right_torque)
  mec_brk_TrailerAxle1_right_torque/1 -> mec_pointmass_generic_ATvoith_std/15(mec_brk_TrailerAxle1_right_torque)
  mec_brk_TrailerAxle2_right_torque/1 -> mec_pointmass_generic_ATvoith_std/17(mec_brk_TrailerAxle2_right_torque)
  mec_pointmass_generic_ATvoith_std/83(mec_brk_Axle1_left_angPos) -> mec_brk_Axle1_left_angPos/1  "mec_brk_Axle1_left_angPos"
  mec_pointmass_generic_ATvoith_std/82(mec_brk_Axle1_left_angAcc) -> mec_brk_Axle1_left_angAcc/1  "mec_brk_Axle1_left_angAcc"
  mec_pointmass_generic_ATvoith_std/84(mec_brk_Axle1_left_angVel) -> mec_brk_Axle1_left_angVel/1  "mec_brk_Axle1_left_angVel"
  mec_pointmass_generic_ATvoith_std/86(mec_brk_Axle1_right_angPos) -> mec_brk_Axle1_right_angPos/1  "mec_brk_Axle1_right_angPos"
  mec_pointmass_generic_ATvoith_std/85(mec_brk_Axle1_right_angAcc) -> mec_brk_Axle1_right_angAcc/1  "mec_brk_Axle1_right_angAcc"
  mec_pointmass_generic_ATvoith_std/87(mec_brk_Axle1_right_angVel) -> mec_brk_Axle1_right_angVel/1  "mec_brk_Axle1_right_angVel"
  mec_pointmass_generic_ATvoith_std/89(mec_brk_Axle2_left_angPos) -> mec_brk_Axle2_left_angPos/1  "mec_brk_Axle2_left_angPos"
  mec_pointmass_generic_ATvoith_std/88(mec_brk_Axle2_left_angAcc) -> mec_brk_Axle2_left_angAcc/1  "mec_brk_Axle2_left_angAcc"
  mec_pointmass_generic_ATvoith_std/90(mec_brk_Axle2_left_angVel) -> mec_brk_Axle2_left_angVel/1  "mec_brk_Axle2_left_angVel"
  mec_pointmass_generic_ATvoith_std/92(mec_brk_Axle2_right_angPos) -> mec_brk_Axle2_right_angPos/1  "mec_brk_Axle2_right_angPos"
  mec_pointmass_generic_ATvoith_std/91(mec_brk_Axle2_right_angAcc) -> mec_brk_Axle2_right_angAcc/1  "mec_brk_Axle2_right_angAcc"
  mec_pointmass_generic_ATvoith_std/93(mec_brk_Axle2_right_angVel) -> mec_brk_Axle2_right_angVel/1  "mec_brk_Axle2_right_angVel"
  mec_pointmass_generic_ATvoith_std/95(mec_brk_Axle3_left_angPos) -> mec_brk_Axle3_left_angPos/1  "mec_brk_Axle3_left_angPos"
  mec_pointmass_generic_ATvoith_std/94(mec_brk_Axle3_left_angAcc) -> mec_brk_Axle3_left_angAcc/1  "mec_brk_Axle3_left_angAcc"
  mec_pointmass_generic_ATvoith_std/96(mec_brk_Axle3_left_angVel) -> mec_brk_Axle3_left_angVel/1  "mec_brk_Axle3_left_angVel"
  mec_pointmass_generic_ATvoith_std/98(mec_brk_Axle3_right_angPos) -> mec_brk_Axle3_right_angPos/1  "mec_brk_Axle3_right_angPos"
  mec_pointmass_generic_ATvoith_std/97(mec_brk_Axle3_right_angAcc) -> mec_brk_Axle3_right_angAcc/1  "mec_brk_Axle3_right_angAcc"
  mec_pointmass_generic_ATvoith_std/99(mec_brk_Axle3_right_angVel) -> mec_brk_Axle3_right_angVel/1  "mec_brk_Axle3_right_angVel"
  mec_pointmass_generic_ATvoith_std/101(mec_brk_Axle4_left_angPos) -> mec_brk_Axle4_left_angPos/1  "mec_brk_Axle4_left_angPos"
  mec_pointmass_generic_ATvoith_std/100(mec_brk_Axle4_left_angAcc) -> mec_brk_Axle4_left_angAcc/1  "mec_brk_Axle4_left_angAcc"
  mec_pointmass_generic_ATvoith_std/102(mec_brk_Axle4_left_angVel) -> mec_brk_Axle4_left_angVel/1  "mec_brk_Axle4_left_angVel"
  mec_pointmass_generic_ATvoith_std/104(mec_brk_Axle4_right_angPos) -> mec_brk_Axle4_right_angPos/1  "mec_brk_Axle4_right_angPos"
  mec_pointmass_generic_ATvoith_std/103(mec_brk_Axle4_right_angAcc) -> mec_brk_Axle4_right_angAcc/1  "mec_brk_Axle4_right_angAcc"
  mec_pointmass_generic_ATvoith_std/105(mec_brk_Axle4_right_angVel) -> mec_brk_Axle4_right_angVel/1  "mec_brk_Axle4_right_angVel"
  mec_pointmass_generic_ATvoith_std/107(mec_brk_TrailerAxle1_left_angPos) -> mec_brk_TrailerAxle1_left_angPos/1  "mec_brk_TrailerAxle1_left_angPos"
  mec_pointmass_generic_ATvoith_std/106(mec_brk_TrailerAxle1_left_angAcc) -> mec_brk_TrailerAxle1_left_angAcc/1  "mec_brk_TrailerAxle1_left_angAcc"
  mec_pointmass_generic_ATvoith_std/108(mec_brk_TrailerAxle1_left_angVel) -> mec_brk_TrailerAxle1_left_angVel/1  "mec_brk_TrailerAxle1_left_angVel"
  mec_pointmass_generic_ATvoith_std/110(mec_brk_TrailerAxle1_right_angPos) -> mec_brk_TrailerAxle1_right_angPos/1  "mec_brk_TrailerAxle1_right_angPos"
  mec_pointmass_generic_ATvoith_std/109(mec_brk_TrailerAxle1_right_angAcc) -> mec_brk_TrailerAxle1_right_angAcc/1  "mec_brk_TrailerAxle1_right_angAcc"
  mec_pointmass_generic_ATvoith_std/111(mec_brk_TrailerAxle1_right_angVel) -> mec_brk_TrailerAxle1_right_angVel/1  "mec_brk_TrailerAxle1_right_angVel"
  mec_pointmass_generic_ATvoith_std/113(mec_brk_TrailerAxle2_left_angPos) -> mec_brk_TrailerAxle2_left_angPos/1  "mec_brk_TrailerAxle2_left_angPos"
  mec_pointmass_generic_ATvoith_std/112(mec_brk_TrailerAxle2_left_angAcc) -> mec_brk_TrailerAxle2_left_angAcc/1  "mec_brk_TrailerAxle2_left_angAcc"
  mec_pointmass_generic_ATvoith_std/114(mec_brk_TrailerAxle2_left_angVel) -> mec_brk_TrailerAxle2_left_angVel/1  "mec_brk_TrailerAxle2_left_angVel"
  mec_pointmass_generic_ATvoith_std/116(mec_brk_TrailerAxle2_right_angPos) -> mec_brk_TrailerAxle2_right_angPos/1  "mec_brk_TrailerAxle2_right_angPos"
  mec_pointmass_generic_ATvoith_std/115(mec_brk_TrailerAxle2_right_angAcc) -> mec_brk_TrailerAxle2_right_angAcc/1  "mec_brk_TrailerAxle2_right_angAcc"
  mec_pointmass_generic_ATvoith_std/117(mec_brk_TrailerAxle2_right_angVel) -> mec_brk_TrailerAxle2_right_angVel/1  "mec_brk_TrailerAxle2_right_angVel"
  mec_pointmass_generic_ATvoith_std/119(mec_brk_TrailerAxle3_left_angPos) -> mec_brk_TrailerAxle3_left_angPos/1  "mec_brk_TrailerAxle3_left_angPos"
  mec_pointmass_generic_ATvoith_std/118(mec_brk_TrailerAxle3_left_angAcc) -> mec_brk_TrailerAxle3_left_angAcc/1  "mec_brk_TrailerAxle3_left_angAcc"
  mec_pointmass_generic_ATvoith_std/120(mec_brk_TrailerAxle3_left_angVel) -> mec_brk_TrailerAxle3_left_angVel/1  "mec_brk_TrailerAxle3_left_angVel"
  mec_pointmass_generic_ATvoith_std/122(mec_brk_TrailerAxle3_right_angPos) -> mec_brk_TrailerAxle3_right_angPos/1  "mec_brk_TrailerAxle3_right_angPos"
  mec_pointmass_generic_ATvoith_std/121(mec_brk_TrailerAxle3_right_angAcc) -> mec_brk_TrailerAxle3_right_angAcc/1  "mec_brk_TrailerAxle3_right_angAcc"
  mec_pointmass_generic_ATvoith_std/123(mec_brk_TrailerAxle3_right_angVel) -> mec_brk_TrailerAxle3_right_angVel/1  "mec_brk_TrailerAxle3_right_angVel"
  mec_brk_TrailerAxle3_left_torque/1 -> mec_pointmass_generic_ATvoith_std/18(mec_brk_TrailerAxle3_left_torque)
  mec_brk_TrailerAxle3_right_torque/1 -> mec_pointmass_generic_ATvoith_std/19(mec_brk_TrailerAxle3_right_torque)
  DIWA_NXT/10(MinRetTrqPwrUp_Stat_PT) -> mec_MinRetTrqPwrUp_Stat_PT/1
  DIWA_NXT/9(RetAct_Stat_PT) -> mec_RetAct_Stat_PT/1
  DIWA_NXT/8(FuncLmpRET_Rq) -> mec_FuncLmpRet_Rq/1
  DIWA_NXT/7(ActMaxRetTrqNoTemp_Cval_PT) -> mec_ActMaxRetTrqNoTemp_Cval_PT/1
  DIWA_NXT/6(MaxRetTrq_Cval_PT) -> mec_MaxRetTrq_Cval_PT/1
  DIWA_NXT/3(Verlustmoment_am_Getriebeeingang_Nm) -> mec_tx_TiLossIn_info/1
  DIWA_NXT/12(n1_rpm) -> mec_tx_n1/1
  DIWA_NXT/11(n2_rpm) -> mec_tx_n2/1
  DIWA_NXT/5(RetTrqCval_PT) -> mec_RetTrqCval_PT/1
  DIWA_NXT/4(BremsmomentBetriebsbremse) -> mec_BrkTrqServBrk_Nm/1
  tcm_p_RGK/1 -> DIWA_NXT/11(tcm_p_RGK)
  pt_RetTrq_Rq_PT/1 -> DIWA_NXT/12(RetTrq_Rq_PT)
  tcm_gearAct/1 -> DIWA_NXT/13(current_gear)
  pt_ReqGr_Stat_PT/1 -> DIWA_NXT/14(requested_gear)
  mec_eng_CrankMean_torque/1 -> Engine/7(mec_eng_CrankMean_torque), Sum1/2
  mec_pointmass_generic_ATvoith_std/146(mec_veh_massVehicle) -> mec_veh_massVehicle/1  "mec_veh_massVehicle"
  mec_pointmass_generic_ATvoith_std/152(mec_veh_transAcc) -> mec_veh_transAcc/1  "mec_veh_transAcc"
  mec_pointmass_generic_ATvoith_std/153(mec_veh_transPos) -> mec_veh_transPos/1  "mec_veh_transPos"
  mec_pointmass_generic_ATvoith_std/154(mec_veh_transVel) -> mec_veh_transVel/1  "mec_veh_transVel"
  mec_pointmass_generic_ATvoith_std/141(mec_veh_AxleLoad1) -> mec_veh_AxleLoad1/1  "mec_veh_AxleLoad1"
  mec_pointmass_generic_ATvoith_std/142(mec_veh_AxleLoad2) -> mec_veh_AxleLoad2/1  "mec_veh_AxleLoad2"
  mec_pointmass_generic_ATvoith_std/143(mec_veh_AxleLoad3) -> mec_veh_AxleLoad3/1  "mec_veh_AxleLoad3"
  mec_pointmass_generic_ATvoith_std/144(mec_veh_AxleLoad4) -> mec_veh_AxleLoad4/1  "mec_veh_AxleLoad4"
  mec_pointmass_generic_ATvoith_std/145(mec_veh_fRollCoeffOverall) -> mec_veh_fRollCoeffOverall/1  "mec_veh_fRollCoeffOverall"
  mec_pointmass_generic_ATvoith_std/147(mec_veh_Payload) -> mec_veh_Payload/1  "mec_veh_Payload"
  mec_pointmass_generic_ATvoith_std/148(mec_veh_TotalGroCombWeight) -> mec_veh_TotalGroCombWeight/1  "mec_veh_TotalGroCombWeight"
  mec_pointmass_generic_ATvoith_std/149(mec_veh_TrailerAxleLoad1) -> mec_veh_TrailerAxleLoad1/1  "mec_veh_TrailerAxleLoad1"
  mec_pointmass_generic_ATvoith_std/150(mec_veh_TrailerAxleLoad2) -> mec_veh_TrailerAxleLoad2/1  "mec_veh_TrailerAxleLoad2"
  mec_pointmass_generic_ATvoith_std/151(mec_veh_TrailerAxleLoad3) -> mec_veh_TrailerAxleLoad3/1  "mec_veh_TrailerAxleLoad3"
  env_load_massdiff/1 -> mec_pointmass_generic_ATvoith_std/4(env_load_massdiff)
